simulink library "ammclib_bam"  (Simulink 9.3)
settings: Solver=VariableStepAuto  StartTime=0.0  StopTime=10.0  RelTol=1e-3
undefined symbols (not defined in the file): f16A1, f16A2, f16ADCMaxError, f16B0, f16B1, f16B2, f16C1, f16CC1, f16CC1sc, f16CC1sc_D, f16CC1sc_Q, f16CC2, f16CC2sc, f16CC2sc_D, f16CC2sc_Q, f16DerivGain, f16EGain, f16FiltCoef, f16HystOff, f16HystOn, f16IGain, f16IntegGain, f16IntegGainFW, f16IntegGainQ, f16Kd, f16Kq, f16Limit, f16LowerLimit, f16LowerLimit_D, f16LowerLimit_Q, f16LowerLimitFW, f16LowerLimitQ, f16ModIndex, f16OutValOff, f16OutValOn, f16PropGain, f16PropGainFW, f16PropGainQ, f16RampDown, f16RampUp, f16UGain, f16UpperLimit, f16UpperLimit_D, f16UpperLimit_Q, f16UpperLimitFW, f16UpperLimitQ, f16WIGain, f32A1, f32A2, f32ADCMaxError, f32B0, f32B1, f32B2, f32C1, f32CC1, f32CC1sc, f32CC1sc_D, f32CC1sc_Q, f32CC2, f32CC2sc ... (+62)
(part 8 of 15)

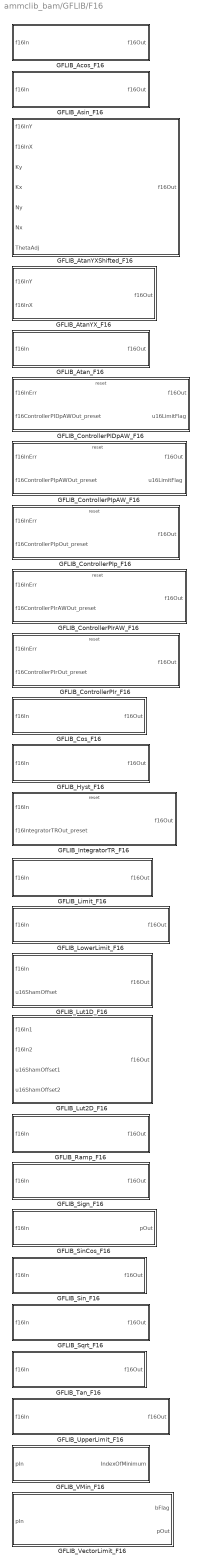
== system ammclib_bam/GFLIB/F16 ==
  GFLIB_Acos_F16 : Subsystem  TreatAsAtomicUnit=on  mask(GFLIB_Acos_F16){}
      mask help: Inverse cosine function in 16-bit fixed-point fractional implementation. Refer to the AMMCLIB User's Guide for further details.
      mask init: same as ammclib_bam/GDFLIB/F16/GDFLIB_FilterFIR_F16
      settings: RTWSystemCode=Inline
      mask Display: pos = get_param(gcb, 'Position');width = pos(3) - pos(1); height = pos(4) - pos(2);tX=width/2;tY=height - 8;color('black');text(tX,tY, 'GFLIB_Acos_F16', 'horizontalAlignment', 'center');
  GFLIB_Asin_F16 : Subsystem  TreatAsAtomicUnit=on  mask(GFLIB_Asin_F16){}
      mask help: Inverse sine function in 16-bit fixed-point fractional implementation. Refer to the AMMCLIB User's Guide for further details.
      mask init: same as ammclib_bam/GDFLIB/F16/GDFLIB_FilterFIR_F16
      settings: RTWSystemCode=Inline
      mask Display: pos = get_param(gcb, 'Position');width = pos(3) - pos(1); height = pos(4) - pos(2);tX=width/2;tY=height - 8;color('black');text(tX,tY, 'GFLIB_Asin_F16', 'horizontalAlignment', 'center');
  GFLIB_AtanYXShifted_F16 : Subsystem  TreatAsAtomicUnit=on  mask(GFLIB_AtanYXShifted_F16){}
      mask help: Shifted arctangent of two arguments Y/X in 16-bit fixed-point fractional implementation. Refer to the AMMCLIB User's Guide for further details.
      mask init: same as ammclib_bam/GDFLIB/F16/GDFLIB_FilterFIR_F16
      settings: RTWSystemCode=Inline
      mask Display: pos = get_param(gcb, 'Position');width = pos(3) - pos(1); height = pos(4) - pos(2);tX=width/2;tY=height - 8;color('black');text(tX,tY, 'GFLIB_AtanYXShifted_F16', 'horizontalAlignment', 'center');
  GFLIB_AtanYX_F16 : Subsystem  TreatAsAtomicUnit=on  mask(GFLIB_AtanYX_F16){}
      mask help: Arctangent of two arguments Y/X in 16-bit fixed-point fractional implementation. Refer to the AMMCLIB User's Guide for further details.
      mask init: same as ammclib_bam/GDFLIB/F16/GDFLIB_FilterFIR_F16
      settings: RTWSystemCode=Inline
      mask Display: pos = get_param(gcb, 'Position');width = pos(3) - pos(1); height = pos(4) - pos(2);tX=width/2;tY=height - 8;color('black');text(tX,tY, 'GFLIB_AtanYX_F16', 'horizontalAlignment', 'center');
  GFLIB_Atan_F16 : Subsystem  TreatAsAtomicUnit=on  mask(GFLIB_Atan_F16){}
      mask help: Inverse tangent function in 16-bit fixed-point fractional implementation. Refer to the AMMCLIB User's Guide for further details.
      mask init: same as ammclib_bam/GDFLIB/F16/GDFLIB_FilterFIR_F16
      settings: RTWSystemCode=Inline
      mask Display: pos = get_param(gcb, 'Position');width = pos(3) - pos(1); height = pos(4) - pos(2);tX=width/2;tY=height - 8;color('black');text(tX,tY, 'GFLIB_Atan_F16', 'horizontalAlignment', 'center');
  GFLIB_ControllerPIDpAW_F16 : Subsystem  TreatAsAtomicUnit=on  mask(GFLIB_ControllerPIDpAW_F16){showStates=Hide (faster execution), resetStatesEnable=Pre-set according to the first set of inputs after reset, f16PropGain=0, f16IntegGain=0, f16DerivGain=0, f16FiltCoef=0, s16PropGainShift=0, s16IntegGainShift=0, s16DerivGainShift=0, f16LowerLimit=0, f16UpperLimit=0}
      mask prompts: showStates "Show internal states"; resetStatesEnable "Internal state after reset"; f16PropGain "f16PropGain (Proportional gain)"; f16IntegGain "f16IntegGain (Integral gain)"; f16DerivGain "f16DerivGain (Derivative gain)"; f16FiltCoef "f16FiltCoef (Derivative term filter coefficient)"; s16PropGainShift "s16PropGainShift (Proportional gain shift)"; s16IntegGainShift "s16IntegGainShift (Integral gain shift)"; s16DerivGainShift "s16DerivGainShift (Derivative gain shift)"; f16LowerLimit "f16LowerLimit (Lower limit of the controller)"; f16UpperLimit "f16UpperLimit (Upper limit of the controller)"
      mask help: Parallel form PID controller with anti-windup in 16-bit fixed-point fractional implementation. This block supports re-initialization of the internal state during simulation. If the block is reset, the controller's output will be aligned with the input f16ControllerPIDpAWOut_preset. Refer to the AMMCLIB User's Guide for further details.
      mask init:
      | if ~evalin('base','exist(''tS8'',''var'')')
      |   if (2 ~= exist('SWLIBS_Typedefs.mat','file'))
      |       error('File SWLIBS_Typedefs.mat is not on the Matlab path. Please add the AMMCLIB "bam" folder in the Matlab Search Path.');
      |   else
      |       evalin('base', 'load(''SWLIBS_Typedefs.mat'')');
      |   end
      | end
      | if showStates == 1
      |     % hidden state variables
      |     if strcmp(get_param([gcb '/f16PropGain'], 'BlockType'), 'Inport')
      |         posblk = get_param(gcb, 'Position');
      | 
      |         pos = get_param(    [gcb, '/f16PropGain'], 'Position');
      |         orient = get_param( [gcb, '/f16PropGain'], 'Orientation');
      |         delete_block(       [gcb, '/f16PropGain']);
      |         add_block('built-in/Ground', [gcb, '/f16PropGain'], 'Position', pos, 'Orientation', orient);
      | 
      |         pos = get_param(    [gcb, '/f16IntegGain'], 'Position');
      |         orient = get_param( [gcb, '/f16IntegGain'], 'Orientation');
      |         delete_block(       [gcb, '/f16IntegGain']);
      |         add_block('built-in/Ground', [gcb, '/f16IntegGain'], 'Position', pos, 'Orientation', orient);
      | 
      |         pos = get_param(    [gcb, '/f16DerivGain'], 'Position');
      |         orient = get_param( [gcb, '/f16DerivGain'], 'Orientation');
      |         delete_block(       [gcb, '/f16DerivGain']);
      |         add_block('built-in/Ground', [gcb, '/f16DerivGain'], 'Position', pos, 'Orientation', orient);
      | 
      |         pos = get_param(    [gcb, '/f16FiltCoef'], 'Position');
      |         orient = get_param( [gcb, '/f16FiltCoef'], 'Orientation');
      |         delete_block(       [gcb, '/f16FiltCoef']);
      |         add_block('built-in/Ground', [gcb, '/f16FiltCoef'], 'Position', pos, 'Orientation', orient);
      | 
      |         pos = get_param(    [gcb, '/s16PropGainShift'], 'Position');
      |         orient = get_param( [gcb, '/s16PropGainShift'], 'Orientation');
      |         delete_block(       [gcb, '/s16PropGainShift']);
      |         add_block('built-in/Ground', [gcb, '/s16PropGainShift'], 'Position', pos, 'Orientation', orient);
      | 
      |         pos = get_param(    [gcb, '/s16IntegGainShift'], 'Position');
      |         orient = get_param( [gcb, '/s16IntegGainShift'], 'Orientation');
      |         delete_block(       [gcb, '/s16IntegGainShift']);
      |         add_block('built-in/Ground', [gcb, '/s16IntegGainShift'], 'Position', pos, 'Orientation', orient);
      | 
      |         pos = get_param(    [gcb, '/s16DerivGainShift'], 'Position');
      |         orient = get_param( [gcb, '/s16DerivGainShift'], 'Orientation');
      |         delete_block(       [gcb, '/s16DerivGainShift']);
      |         add_block('built-in/Ground', [gcb, '/s16DerivGainShift'], 'Position', pos, 'Orientation', orient);
      | 
      |         pos = get_param(    [gcb, '/f16LowerLimit'], 'Position');
      |         orient = get_param( [gcb, '/f16LowerLimit'], 'Orientation');
      |         delete_block(       [gcb, '/f16LowerLimit']);
      |         add_block('built-in/Ground', [gcb, '/f16LowerLimit'], 'Position', pos, 'Orientation', orient);
      | 
      |         pos = get_param(    [gcb, '/f16UpperLimit'], 'Position');
      |         orient = get_param( [gcb, '/f16UpperLimit'], 'Orientation');
      |         delete_block(       [gcb, '/f16UpperLimit']);
      |         add_block('built-in/Ground', [gcb, '/f16UpperLimit'], 'Position', pos, 'Orientation', orient);
      | 
      |         pos = get_param(    [gcb, '/f32IntegPartK_1'], 'Position');
      |         orient = get_param( [gcb, '/f32IntegPartK_1'], 'Orientation');
      |         delete_block(       [gcb, '/f32IntegPartK_1']);
      |         add_block('built-in/Ground', [gcb, '/f32IntegPartK_1'], 'Position', pos, 'Orientation', orient);
      | 
      |         pos = get_param(    [gcb, '/f16DerivPartK_1'], 'Position');
      |         orient = get_param( [gcb, '/f16DerivPartK_1'], 'Orientation');
      |         delete_block(       [gcb, '/f16DerivPartK_1']);
      |         add_block('built-in/Ground', [gcb, '/f16DerivPartK_1'], 'Position', pos, 'Orientation', orient);
      | 
      |         pos = get_param(    [gcb, '/f16InK_1'], 'Position');
      |         orient = get_param( [gcb, '/f16InK_1'], 'Orientation');
      |         delete_block(       [gcb, '/f16InK_1']);
      |         add_block('built-in/Ground', [gcb, '/f16InK_1'], 'Position', pos, 'Orientation', orient);
      | 
      | 
      |         pos = get_param(    [gcb '/f32IntegPartK_1_Out'], 'Position');
      |         orient = get_param( [gcb '/f32IntegPartK_1_Out'], 'Orientation');
      |         delete_block(       [gcb '/f32IntegPartK_1_Out']);
      |         add_block('built-in/Terminator', [gcb '/f32IntegPartK_1_Out'], 'Position', pos, 'Orientation', orient);
      | 
      |         pos = get_param(    [gcb '/f16DerivPartK_1_Out'], 'Position');
      |         orient = get_param( [gcb '/f16DerivPartK_1_Out'], 'Orientation');
      |         delete_block(       [gcb '/f16DerivPartK_1_Out']);
      |         add_block('built-in/Terminator', [gcb '/f16DerivPartK_1_Out'], 'Position', pos, 'Orientation', orient);
      | 
      |         pos = get_param(    [gcb '/f16InK_1_Out'], 'Position');
      |         orient = get_param( [gcb '/f16InK_1_Out'], 'Orientation');
      |         delete_block(       [gcb '/f16InK_1_Out']);
      |         add_block('built-in/Terminator', [gcb '/f16InK_1_Out'], 'Position', pos, 'Orientation', orient);
      | 
      | 
      |         set_param([gcb '/f16InErr'], 'Port', '1');
      |         set_param([gcb '/f16ControllerPIDpAWOut_preset'], 'Port', '2');
      | 
      |         set_param([gcb '/f16Out'], 'Port', '1');
      |         set_param([gcb '/u16LimitFlag'], 'Port', '2');
      | 
      |         set_param(gcb,'MaskEnables',{'on','on','on','on','on','on','on','on','on','on','on'});
      | 
      |         if (posblk(4) - posblk(2)) > 75
      |           height = 75;
      |           set_param(gcb,'Position',[posblk(1), posblk(2), posblk(3), posblk(2)+height])
      |         end
      |     end
      | else
      |     % shown state variables
      |     if strcmp(get_param([gcb '/f16PropGain'], 'BlockType'), 'Ground')
      |         posblk = get_param(gcb, 'Position');
      | 
      |         pos = get_param(    [gcb, '/f16PropGain'], 'Position');
      |         orient = get_param( [gcb, '/f16PropGain'], 'Orientation');
      |         delete_block(       [gcb, '/f16PropGain']);
      |         add_block('built-in/Inport', [gcb, '/f16PropGain'], 'Position', pos, 'Orientation', orient, 'OutDataTypeStr', 'int16');
      | 
      |         pos = get_param(    [gcb, '/f16IntegGain'], 'Position');
      |         orient = get_param( [gcb, '/f16IntegGain'], 'Orientation');
      |         delete_block(       [gcb, '/f16IntegGain']);
      |         add_block('built-in/Inport', [gcb, '/f16IntegGain'], 'Position', pos, 'Orientation', orient, 'OutDataTypeStr', 'int16');
      | 
      |         pos = get_param(    [gcb, '/f16DerivGain'], 'Position');
      |         orient = get_param( [gcb, '/f16DerivGain'], 'Orientation');
      |         delete_block(       [gcb, '/f16DerivGain']);
      |         add_block('built-in/Inport', [gcb, '/f16DerivGain'], 'Position', pos, 'Orientation', orient, 'OutDataTypeStr', 'int16');
      | 
      |         pos = get_param(    [gcb, '/f16FiltCoef'], 'Position');
      |         orient = get_param( [gcb, '/f16FiltCoef'], 'Orientation');
      |         delete_block(       [gcb, '/f16FiltCoef']);
      |         add_block('built-in/Inport', [gcb, '/f16FiltCoef'], 'Position', pos, 'Orientation', orient, 'OutDataTypeStr', 'int16');
      | 
      |         pos = get_param(    [gcb, '/s16PropGainShift'], 'Position');
      |         orient = get_param( [gcb, '/s16PropGainShift'], 'Orientation');
      |         delete_block(       [gcb, '/s16PropGainShift']);
      |         add_block('built-in/Inport', [gcb, '/s16PropGainShift'], 'Position', pos, 'Orientation', orient, 'OutDataTypeStr', 'int16');
      | 
      |         pos = get_param(    [gcb, '/s16IntegGainShift'], 'Position');
      |         orient = get_param( [gcb, '/s16IntegGainShift'], 'Orientation');
      |         delete_block(       [gcb, '/s16IntegGainShift']);
      |         add_block('built-in/Inport', [gcb, '/s16IntegGainShift'], 'Position', pos, 'Orientation', orient, 'OutDataTypeStr', 'int16');
      | 
      |         pos = get_param(    [gcb, '/s16DerivGainShift'], 'Position');
      |         orient = get_param( [gcb, '/s16DerivGainShift'], 'Orientation');
      |         delete_block(       [gcb, '/s16DerivGainShift']);
      |         add_block('built-in/Inport', [gcb, '/s16DerivGainShift'], 'Position', pos, 'Orientation', orient, 'OutDataTypeStr', 'int16');
      | 
      |         pos = get_param(    [gcb, '/f16LowerLimit'], 'Position');
      |         orient = get_param( [gcb, '/f16LowerLimit'], 'Orientation');
      |         delete_block(       [gcb, '/f16LowerLimit']);
      |         add_block('built-in/Inport', [gcb, '/f16LowerLimit'], 'Position', pos, 'Orientation', orient, 'OutDataTypeStr', 'int16');
      | 
      |         pos = get_param(    [gcb, '/f16UpperLimit'], 'Position');
      |         orient = get_param( [gcb, '/f16UpperLimit'], 'Orientation');
      |         delete_block(       [gcb, '/f16UpperLimit']);
      |         add_block('built-in/Inport', [gcb, '/f16UpperLimit'], 'Position', pos, 'Orientation', orient, 'OutDataTypeStr', 'int16');
      | 
      |         pos = get_param(    [gcb, '/f32IntegPartK_1'], 'Position');
      |         orient = get_param( [gcb, '/f32IntegPartK_1'], 'Orientation');
      |         delete_block(       [gcb, '/f32IntegPartK_1']);
      |         add_block('built-in/Inport', [gcb, '/f32IntegPartK_1'], 'Position', pos, 'Orientation', orient, 'OutDataTypeStr', 'int32');
      | 
      |         pos = get_param(    [gcb, '/f16DerivPartK_1'], 'Position');
      |         orient = get_param( [gcb, '/f16DerivPartK_1'], 'Orientation');
      |         delete_block(       [gcb, '/f16DerivPartK_1']);
      |         add_block('built-in/Inport', [gcb, '/f16DerivPartK_1'], 'Position', pos, 'Orientation', orient, 'OutDataTypeStr', 'int16');
      | 
      |         pos = get_param(    [gcb, '/f16InK_1'], 'Position');
      |         orient = get_param( [gcb, '/f16InK_1'], 'Orientation');
      |         delete_block(       [gcb, '/f16InK_1']);
      |         add_block('built-in/Inport', [gcb, '/f16InK_1'], 'Position', pos, 'Orientation', orient, 'OutDataTypeStr', 'int16');
      | 
      | 
      |         pos = get_param(    [gcb '/f32IntegPartK_1_Out'], 'Position');
      |         orient = get_param( [gcb '/f32IntegPartK_1_Out'], 'Orientation');
      |         delete_block(       [gcb '/f32IntegPartK_1_Out']);
      |         add_block('built-in/Outport', [gcb '/f32IntegPartK_1_Out'], 'Position', pos, 'Orientation', orient);
      | 
      |         pos = get_param(    [gcb '/f16DerivPartK_1_Out'], 'Position');
      |         orient = get_param( [gcb '/f16DerivPartK_1_Out'], 'Orientation');
      |         delete_block(       [gcb '/f16DerivPartK_1_Out']);
      |         add_block('built-in/Outport', [gcb '/f16DerivPartK_1_Out'], 'Position', pos, 'Orientation', orient);
      | 
      |         pos = get_param(    [gcb '/f16InK_1_Out'], 'Position');
      |         orient = get_param( [gcb '/f16InK_1_Out'], 'Orientation');
      |         delete_block(       [gcb '/f16InK_1_Out']);
      |         add_block('built-in/Outport', [gcb '/f16InK_1_Out'], 'Position', pos, 'Orientation', orient);
      | 
      | 
      |         set_param([gcb '/f16InErr'], 'Port', '1');
      |         set_param([gcb '/f16ControllerPIDpAWOut_preset'], 'Port', '2');
      |         set_param([gcb '/f16PropGain'], 'Port', '3');
      |         set_param([gcb '/f16IntegGain'], 'Port', '4');
      |         set_param([gcb '/f16DerivGain'], 'Port', '5');
      |         set_param([gcb '/f16FiltCoef'], 'Port', '6');
      |         set_param([gcb '/s16PropGainShift'], 'Port', '7');
      |         set_param([gcb '/s16IntegGainShift'], 'Port', '8');
      |         set_param([gcb '/s16DerivGainShift'], 'Port', '9');
      |         set_param([gcb '/f16LowerLimit'], 'Port', '10');
      |         set_param([gcb '/f16UpperLimit'], 'Port', '11');
      |         set_param([gcb '/f32IntegPartK_1'], 'Port', '12');
      |         set_param([gcb '/f16DerivPartK_1'], 'Port', '13');
      |         set_param([gcb '/f16InK_1'], 'Port', '14');
      | 
      |         set_param([gcb '/f16Out'], 'Port', '1');
      |         set_param([gcb '/u16LimitFlag'], 'Port', '2');
      |         set_param([gcb '/f32IntegPartK_1_Out'], 'Port', '3');
      |         set_param([gcb '/f16DerivPartK_1_Out'], 'Port', '4');
      |         set_param([gcb '/f16InK_1_Out'], 'Port', '5');
      | 
      |         set_param(gcb,'MaskEnables',{'on','on','off','off','off','off','off','off','off','off','off'});
      | 
      |         if (posblk(4) - posblk(2)) < 375
      |           height = 375;
      |           set_param(gcb,'Position',[posblk(1), posblk(2), posblk(3), posblk(2)+height])
      |         end
      |     end
      | end
      settings: RTWSystemCode=Inline
      mask TypeOptions showStates: Hide (faster execution) | Show (allows debugging; connect feedback loops manually)
      mask Callback showStates:
      | maskStr = get_param(gcb,'showStates');
      | if strcmp(maskStr,'Hide (faster execution)'),
      |     set_param(gcb,'MaskEnables',{'on','on','on','on','on','on','on','on','on','on','on'});
      | else
      |     set_param(gcb,'MaskEnables',{'on','on','off','off','off','off','off','off','off','off','off'});
      | end
      mask TypeOptions resetStatesEnable: Pre-set according to the first set of inputs after reset | Clear to zero
      mask Display:
      | color('black');
      | pos = get_param(gcb, 'Position');
      | width = pos(3) - pos(1);
      | height = pos(4) - pos(2);
      | tX=width/2;
      | tY=height - 25;
      | color('black');
      | text(tX,tY, 'GFLIB_ControllerPIDpAW_F16', 'horizontalAlignment', 'center');
      | if showStates == 2
      |   color('red');
      |   text(tX,tY - 20, ['debugging mode' char(13) char(10) '(limited performance)'], 'horizontalAlignment', 'center');
      | end
  GFLIB_ControllerPIpAW_F16 : Subsystem  TreatAsAtomicUnit=on  mask(GFLIB_ControllerPIpAW_F16){showStates=Hide (faster execution), resetStatesEnable=Pre-set according to the first set of inputs after reset, f16PropGain=0, f16IntegGain=0, s16PropGainShift=0, s16IntegGainShift=0, f16LowerLimit=0, f16UpperLimit=0}
      mask prompts: showStates "Show internal states"; resetStatesEnable "Internal state after reset"; f16PropGain "f16PropGain (Proportional gain)"; f16IntegGain "f16IntegGain (Integral gain)"; s16PropGainShift "s16PropGainShift (Proportional gain shift)"; s16IntegGainShift "s16IntegGainShift (Integral gain shift)"; f16LowerLimit "f16LowerLimit (Lower limit of the controller)"; f16UpperLimit "f16UpperLimit (Upper limit of the controller)"
      mask help: Parallel form PI controller with anti-windup in 16-bit fixed-point fractional implementation. This block supports re-initialization of the internal state during simulation. If the block is reset, the controller's output will be aligned with the input f16ControllerPIpAWOut_preset. Refer to the AMMCLIB User's Guide for further details.
      mask init:
      | if ~evalin('base','exist(''tS8'',''var'')')
      |   if (2 ~= exist('SWLIBS_Typedefs.mat','file'))
      |       error('File SWLIBS_Typedefs.mat is not on the Matlab path. Please add the AMMCLIB "bam" folder in the Matlab Search Path.');
      |   else
      |       evalin('base', 'load(''SWLIBS_Typedefs.mat'')');
      |   end
      | end
      | if showStates == 1
      |     % hidden state variables
      |     if strcmp(get_param([gcb '/f16PropGain'], 'BlockType'), 'Inport')
      |         posblk = get_param(gcb, 'Position');
      | 
      |         pos = get_param(    [gcb, '/f16PropGain'], 'Position');
      |         orient = get_param( [gcb, '/f16PropGain'], 'Orientation');
      |         delete_block(       [gcb, '/f16PropGain']);
      |         add_block('built-in/Ground', [gcb, '/f16PropGain'], 'Position', pos, 'Orientation', orient);
      | 
      |         pos = get_param(    [gcb, '/f16IntegGain'], 'Position');
      |         orient = get_param( [gcb, '/f16IntegGain'], 'Orientation');
      |         delete_block(       [gcb, '/f16IntegGain']);
      |         add_block('built-in/Ground', [gcb, '/f16IntegGain'], 'Position', pos, 'Orientation', orient);
      | 
      |         pos = get_param(    [gcb, '/s16PropGainShift'], 'Position');
      |         orient = get_param( [gcb, '/s16PropGainShift'], 'Orientation');
      |         delete_block(       [gcb, '/s16PropGainShift']);
      |         add_block('built-in/Ground', [gcb, '/s16PropGainShift'], 'Position', pos, 'Orientation', orient);
      | 
      |         pos = get_param(    [gcb, '/s16IntegGainShift'], 'Position');
      |         orient = get_param( [gcb, '/s16IntegGainShift'], 'Orientation');
      |         delete_block(       [gcb, '/s16IntegGainShift']);
      |         add_block('built-in/Ground', [gcb, '/s16IntegGainShift'], 'Position', pos, 'Orientation', orient);
      | 
      |         pos = get_param(    [gcb, '/f16LowerLimit'], 'Position');
      |         orient = get_param( [gcb, '/f16LowerLimit'], 'Orientation');
      |         delete_block(       [gcb, '/f16LowerLimit']);
      |         add_block('built-in/Ground', [gcb, '/f16LowerLimit'], 'Position', pos, 'Orientation', orient);
      | 
      |         pos = get_param(    [gcb, '/f16UpperLimit'], 'Position');
      |         orient = get_param( [gcb, '/f16UpperLimit'], 'Orientation');
      |         delete_block(       [gcb, '/f16UpperLimit']);
      |         add_block('built-in/Ground', [gcb, '/f16UpperLimit'], 'Position', pos, 'Orientation', orient);
      | 
      |         pos = get_param(    [gcb, '/f32IntegPartK_1'], 'Position');
      |         orient = get_param( [gcb, '/f32IntegPartK_1'], 'Orientation');
      |         delete_block(       [gcb, '/f32IntegPartK_1']);
      |         add_block('built-in/Ground', [gcb, '/f32IntegPartK_1'], 'Position', pos, 'Orientation', orient);
      | 
      |         pos = get_param(    [gcb, '/f16InK_1'], 'Position');
      |         orient = get_param( [gcb, '/f16InK_1'], 'Orientation');
      |         delete_block(       [gcb, '/f16InK_1']);
      |         add_block('built-in/Ground', [gcb, '/f16InK_1'], 'Position', pos, 'Orientation', orient);
      | 
      | 
      |         pos = get_param(    [gcb '/f32IntegPartK_1_Out'], 'Position');
      |         orient = get_param( [gcb '/f32IntegPartK_1_Out'], 'Orientation');
      |         delete_block(       [gcb '/f32IntegPartK_1_Out']);
      |         add_block('built-in/Terminator', [gcb '/f32IntegPartK_1_Out'], 'Position', pos, 'Orientation', orient);
      | 
      |         pos = get_param(    [gcb '/f16InK_1_Out'], 'Position');
      |         orient = get_param( [gcb '/f16InK_1_Out'], 'Orientation');
      |         delete_block(       [gcb '/f16InK_1_Out']);
      |         add_block('built-in/Terminator', [gcb '/f16InK_1_Out'], 'Position', pos, 'Orientation', orient);
      | 
      | 
      |         set_param([gcb '/f16InErr'], 'Port', '1');
      |         set_param([gcb '/f16ControllerPIpAWOut_preset'], 'Port', '2');
      | 
      |         set_param([gcb '/f16Out'], 'Port', '1');
      |         set_param([gcb '/u16LimitFlag'], 'Port', '2');
      | 
      |         set_param(gcb,'MaskEnables',{'on','on','on','on','on','on','on','on'});
      | 
      |         if (posblk(4) - posblk(2)) > 75
      |           height = 75;
      |           set_param(gcb,'Position',[posblk(1), posblk(2), posblk(3), posblk(2)+height])
      |         end
      |     end
      | else
      |     % shown state variables
      |     if strcmp(get_param([gcb '/f16PropGain'], 'BlockType'), 'Ground')
      |         posblk = get_param(gcb, 'Position');
      | 
      |         pos = get_param(    [gcb, '/f16PropGain'], 'Position');
      |         orient = get_param( [gcb, '/f16PropGain'], 'Orientation');
      |         delete_block(       [gcb, '/f16PropGain']);
      |         add_block('built-in/Inport', [gcb, '/f16PropGain'], 'Position', pos, 'Orientation', orient, 'OutDataTypeStr', 'int16');
      | 
      |         pos = get_param(    [gcb, '/f16IntegGain'], 'Position');
      |         orient = get_param( [gcb, '/f16IntegGain'], 'Orientation');
      |         delete_block(       [gcb, '/f16IntegGain']);
      |         add_block('built-in/Inport', [gcb, '/f16IntegGain'], 'Position', pos, 'Orientation', orient, 'OutDataTypeStr', 'int16');
      | 
      |         pos = get_param(    [gcb, '/s16PropGainShift'], 'Position');
      |         orient = get_param( [gcb, '/s16PropGainShift'], 'Orientation');
      |         delete_block(       [gcb, '/s16PropGainShift']);
      |         add_block('built-in/Inport', [gcb, '/s16PropGainShift'], 'Position', pos, 'Orientation', orient, 'OutDataTypeStr', 'int16');
      | 
      |         pos = get_param(    [gcb, '/s16IntegGainShift'], 'Position');
      |         orient = get_param( [gcb, '/s16IntegGainShift'], 'Orientation');
      |         delete_block(       [gcb, '/s16IntegGainShift']);
      |         add_block('built-in/Inport', [gcb, '/s16IntegGainShift'], 'Position', pos, 'Orientation', orient, 'OutDataTypeStr', 'int16');
      | 
      |         pos = get_param(    [gcb, '/f16LowerLimit'], 'Position');
      |         orient = get_param( [gcb, '/f16LowerLimit'], 'Orientation');
      |         delete_block(       [gcb, '/f16LowerLimit']);
      |         add_block('built-in/Inport', [gcb, '/f16LowerLimit'], 'Position', pos, 'Orientation', orient, 'OutDataTypeStr', 'int16');
      | 
      |         pos = get_param(    [gcb, '/f16UpperLimit'], 'Position');
      |         orient = get_param( [gcb, '/f16UpperLimit'], 'Orientation');
      |         delete_block(       [gcb, '/f16UpperLimit']);
      |         add_block('built-in/Inport', [gcb, '/f16UpperLimit'], 'Position', pos, 'Orientation', orient, 'OutDataTypeStr', 'int16');
      | 
      |         pos = get_param(    [gcb, '/f32IntegPartK_1'], 'Position');
      |         orient = get_param( [gcb, '/f32IntegPartK_1'], 'Orientation');
      |         delete_block(       [gcb, '/f32IntegPartK_1']);
      |         add_block('built-in/Inport', [gcb, '/f32IntegPartK_1'], 'Position', pos, 'Orientation', orient, 'OutDataTypeStr', 'int32');
      | 
      |         pos = get_param(    [gcb, '/f16InK_1'], 'Position');
      |         orient = get_param( [gcb, '/f16InK_1'], 'Orientation');
      |         delete_block(       [gcb, '/f16InK_1']);
      |         add_block('built-in/Inport', [gcb, '/f16InK_1'], 'Position', pos, 'Orientation', orient, 'OutDataTypeStr', 'int16');
      | 
      | 
      |         pos = get_param(    [gcb '/f32IntegPartK_1_Out'], 'Position');
      |         orient = get_param( [gcb '/f32IntegPartK_1_Out'], 'Orientation');
      |         delete_block(       [gcb '/f32IntegPartK_1_Out']);
      |         add_block('built-in/Outport', [gcb '/f32IntegPartK_1_Out'], 'Position', pos, 'Orientation', orient);
      | 
      |         pos = get_param(    [gcb '/f16InK_1_Out'], 'Position');
      |         orient = get_param( [gcb '/f16InK_1_Out'], 'Orientation');
      |         delete_block(       [gcb '/f16InK_1_Out']);
      |         add_block('built-in/Outport', [gcb '/f16InK_1_Out'], 'Position', pos, 'Orientation', orient);
      | 
      | 
      |         set_param([gcb '/f16InErr'], 'Port', '1');
      |         set_param([gcb '/f16ControllerPIpAWOut_preset'], 'Port', '2');
      |         set_param([gcb '/f16PropGain'], 'Port', '3');
      |         set_param([gcb '/f16IntegGain'], 'Port', '4');
      |         set_param([gcb '/s16PropGainShift'], 'Port', '5');
      |         set_param([gcb '/s16IntegGainShift'], 'Port', '6');
      |         set_param([gcb '/f16LowerLimit'], 'Port', '7');
      |         set_param([gcb '/f16UpperLimit'], 'Port', '8');
      |         set_param([gcb '/f32IntegPartK_1'], 'Port', '9');
      |         set_param([gcb '/f16InK_1'], 'Port', '10');
      | 
      |         set_param([gcb '/f16Out'], 'Port', '1');
      |         set_param([gcb '/u16LimitFlag'], 'Port', '2');
      |         set_param([gcb '/f32IntegPartK_1_Out'], 'Port', '3');
      |         set_param([gcb '/f16InK_1_Out'], 'Port', '4');
      | 
      |         set_param(gcb,'MaskEnables',{'on','on','off','off','off','off','off','off'});
      | 
      |         if (posblk(4) - posblk(2)) < 275
      |           height = 275;
      |           set_param(gcb,'Position',[posblk(1), posblk(2), posblk(3), posblk(2)+height])
      |         end
      |     end
      | end
      settings: RTWSystemCode=Inline
      mask TypeOptions showStates: Hide (faster execution) | Show (allows debugging; connect feedback loops manually)
      mask Callback showStates:
      | maskStr = get_param(gcb,'showStates');
      | if strcmp(maskStr,'Hide (faster execution)'),
      |     set_param(gcb,'MaskEnables',{'on','on','on','on','on','on','on','on'});
      | else
      |     set_param(gcb,'MaskEnables',{'on','on','off','off','off','off','off','off'});
      | end
      mask TypeOptions resetStatesEnable: Pre-set according to the first set of inputs after reset | Clear to zero
      mask Display:
      | color('black');
      | pos = get_param(gcb, 'Position');
      | width = pos(3) - pos(1);
      | height = pos(4) - pos(2);
      | tX=width/2;
      | tY=height - 25;
      | color('black');
      | text(tX,tY, 'GFLIB_ControllerPIpAW_F16', 'horizontalAlignment', 'center');
      | if showStates == 2
      |   color('red');
      |   text(tX,tY - 20, ['debugging mode' char(13) char(10) '(limited performance)'], 'horizontalAlignment', 'center');
      | end
  GFLIB_ControllerPIp_F16 : Subsystem  TreatAsAtomicUnit=on  mask(GFLIB_ControllerPIp_F16){showStates=Hide (faster execution), resetStatesEnable=Pre-set according to the first set of inputs after reset, f16PropGain=0, f16IntegGain=0, s16PropGainShift=0, s16IntegGainShift=0}
      mask prompts: showStates "Show internal states"; resetStatesEnable "Internal state after reset"; f16PropGain "f16PropGain (Proportional gain)"; f16IntegGain "f16IntegGain (Integral gain)"; s16PropGainShift "s16PropGainShift (Proportional gain shift)"; s16IntegGainShift "s16IntegGainShift (Integral gain shift)"
      mask help: Parallel form PI controller without anti-windup in 16-bit fixed-point fractional implementation. This block supports re-initialization of the internal state during simulation. If the block is reset, the controller's output will be aligned with the input f16ControllerPIpOut_preset. Refer to the AMMCLIB User's Guide for further details.
      mask init:
      | if ~evalin('base','exist(''tS8'',''var'')')
      |   if (2 ~= exist('SWLIBS_Typedefs.mat','file'))
      |       error('File SWLIBS_Typedefs.mat is not on the Matlab path. Please add the AMMCLIB "bam" folder in the Matlab Search Path.');
      |   else
      |       evalin('base', 'load(''SWLIBS_Typedefs.mat'')');
      |   end
      | end
      | if showStates == 1
      |     % hidden state variables
      |     if strcmp(get_param([gcb '/f16PropGain'], 'BlockType'), 'Inport')
      |         posblk = get_param(gcb, 'Position');
      | 
      |         pos = get_param(    [gcb, '/f16PropGain'], 'Position');
      |         orient = get_param( [gcb, '/f16PropGain'], 'Orientation');
      |         delete_block(       [gcb, '/f16PropGain']);
      |         add_block('built-in/Ground', [gcb, '/f16PropGain'], 'Position', pos, 'Orientation', orient);
      | 
      |         pos = get_param(    [gcb, '/f16IntegGain'], 'Position');
      |         orient = get_param( [gcb, '/f16IntegGain'], 'Orientation');
      |         delete_block(       [gcb, '/f16IntegGain']);
      |         add_block('built-in/Ground', [gcb, '/f16IntegGain'], 'Position', pos, 'Orientation', orient);
      | 
      |         pos = get_param(    [gcb, '/s16PropGainShift'], 'Position');
      |         orient = get_param( [gcb, '/s16PropGainShift'], 'Orientation');
      |         delete_block(       [gcb, '/s16PropGainShift']);
      |         add_block('built-in/Ground', [gcb, '/s16PropGainShift'], 'Position', pos, 'Orientation', orient);
      | 
      |         pos = get_param(    [gcb, '/s16IntegGainShift'], 'Position');
      |         orient = get_param( [gcb, '/s16IntegGainShift'], 'Orientation');
      |         delete_block(       [gcb, '/s16IntegGainShift']);
      |         add_block('built-in/Ground', [gcb, '/s16IntegGainShift'], 'Position', pos, 'Orientation', orient);
      | 
      |         pos = get_param(    [gcb, '/f32IntegPartK_1'], 'Position');
      |         orient = get_param( [gcb, '/f32IntegPartK_1'], 'Orientation');
      |         delete_block(       [gcb, '/f32IntegPartK_1']);
      |         add_block('built-in/Ground', [gcb, '/f32IntegPartK_1'], 'Position', pos, 'Orientation', orient);
      | 
      |         pos = get_param(    [gcb, '/f16InK_1'], 'Position');
      |         orient = get_param( [gcb, '/f16InK_1'], 'Orientation');
      |         delete_block(       [gcb, '/f16InK_1']);
      |         add_block('built-in/Ground', [gcb, '/f16InK_1'], 'Position', pos, 'Orientation', orient);
      | 
      | 
      |         pos = get_param(    [gcb '/f32IntegPartK_1_Out'], 'Position');
      |         orient = get_param( [gcb '/f32IntegPartK_1_Out'], 'Orientation');
      |         delete_block(       [gcb '/f32IntegPartK_1_Out']);
      |         add_block('built-in/Terminator', [gcb '/f32IntegPartK_1_Out'], 'Position', pos, 'Orientation', orient);
      | 
      |         pos = get_param(    [gcb '/f16InK_1_Out'], 'Position');
      |         orient = get_param( [gcb '/f16InK_1_Out'], 'Orientation');
      |         delete_block(       [gcb '/f16InK_1_Out']);
      |         add_block('built-in/Terminator', [gcb '/f16InK_1_Out'], 'Position', pos, 'Orientation', orient);
      | 
      | 
      |         set_param([gcb '/f16InErr'], 'Port', '1');
      |         set_param([gcb '/f16ControllerPIpOut_preset'], 'Port', '2');
      | 
      |         set_param([gcb '/f16Out'], 'Port', '1');
      | 
      |         set_param(gcb,'MaskEnables',{'on','on','on','on','on','on'});
      | 
      |         if (posblk(4) - posblk(2)) > 75
      |           height = 75;
      |           set_param(gcb,'Position',[posblk(1), posblk(2), posblk(3), posblk(2)+height])
      |         end
      |     end
      | else
      |     % shown state variables
      |     if strcmp(get_param([gcb '/f16PropGain'], 'BlockType'), 'Ground')
      |         posblk = get_param(gcb, 'Position');
      | 
      |         pos = get_param(    [gcb, '/f16PropGain'], 'Position');
      |         orient = get_param( [gcb, '/f16PropGain'], 'Orientation');
      |         delete_block(       [gcb, '/f16PropGain']);
      |         add_block('built-in/Inport', [gcb, '/f16PropGain'], 'Position', pos, 'Orientation', orient, 'OutDataTypeStr', 'int16');
      | 
      |         pos = get_param(    [gcb, '/f16IntegGain'], 'Position');
      |         orient = get_param( [gcb, '/f16IntegGain'], 'Orientation');
      |         delete_block(       [gcb, '/f16IntegGain']);
      |         add_block('built-in/Inport', [gcb, '/f16IntegGain'], 'Position', pos, 'Orientation', orient, 'OutDataTypeStr', 'int16');
      | 
      |         pos = get_param(    [gcb, '/s16PropGainShift'], 'Position');
      |         orient = get_param( [gcb, '/s16PropGainShift'], 'Orientation');
      |         delete_block(       [gcb, '/s16PropGainShift']);
      |         add_block('built-in/Inport', [gcb, '/s16PropGainShift'], 'Position', pos, 'Orientation', orient, 'OutDataTypeStr', 'int16');
      | 
      |         pos = get_param(    [gcb, '/s16IntegGainShift'], 'Position');
      |         orient = get_param( [gcb, '/s16IntegGainShift'], 'Orientation');
      |         delete_block(       [gcb, '/s16IntegGainShift']);
      |         add_block('built-in/Inport', [gcb, '/s16IntegGainShift'], 'Position', pos, 'Orientation', orient, 'OutDataTypeStr', 'int16');
      | 
      |         pos = get_param(    [gcb, '/f32IntegPartK_1'], 'Position');
      |         orient = get_param( [gcb, '/f32IntegPartK_1'], 'Orientation');
      |         delete_block(       [gcb, '/f32IntegPartK_1']);
      |         add_block('built-in/Inport', [gcb, '/f32IntegPartK_1'], 'Position', pos, 'Orientation', orient, 'OutDataTypeStr', 'int32');
      | 
      |         pos = get_param(    [gcb, '/f16InK_1'], 'Position');
      |         orient = get_param( [gcb, '/f16InK_1'], 'Orientation');
      |         delete_block(       [gcb, '/f16InK_1']);
      |         add_block('built-in/Inport', [gcb, '/f16InK_1'], 'Position', pos, 'Orientation', orient, 'OutDataTypeStr', 'int16');
      | 
      | 
      |         pos = get_param(    [gcb '/f32IntegPartK_1_Out'], 'Position');
      |         orient = get_param( [gcb '/f32IntegPartK_1_Out'], 'Orientation');
      |         delete_block(       [gcb '/f32IntegPartK_1_Out']);
      |         add_block('built-in/Outport', [gcb '/f32IntegPartK_1_Out'], 'Position', pos, 'Orientation', orient);
      | 
      |         pos = get_param(    [gcb '/f16InK_1_Out'], 'Position');
      |         orient = get_param( [gcb '/f16InK_1_Out'], 'Orientation');
      |         delete_block(       [gcb '/f16InK_1_Out']);
      |         add_block('built-in/Outport', [gcb '/f16InK_1_Out'], 'Position', pos, 'Orientation', orient);
      | 
      | 
      |         set_param([gcb '/f16InErr'], 'Port', '1');
      |         set_param([gcb '/f16ControllerPIpOut_preset'], 'Port', '2');
      |         set_param([gcb '/f16PropGain'], 'Port', '3');
      |         set_param([gcb '/f16IntegGain'], 'Port', '4');
      |         set_param([gcb '/s16PropGainShift'], 'Port', '5');
      |         set_param([gcb '/s16IntegGainShift'], 'Port', '6');
      |         set_param([gcb '/f32IntegPartK_1'], 'Port', '7');
      |         set_param([gcb '/f16InK_1'], 'Port', '8');
      | 
      |         set_param([gcb '/f16Out'], 'Port', '1');
      |         set_param([gcb '/f32IntegPartK_1_Out'], 'Port', '2');
      |         set_param([gcb '/f16InK_1_Out'], 'Port', '3');
      | 
      |         set_param(gcb,'MaskEnables',{'on','on','off','off','off','off'});
      | 
      |         if (posblk(4) - posblk(2)) < 225
      |           height = 225;
      |           set_param(gcb,'Position',[posblk(1), posblk(2), posblk(3), posblk(2)+height])
      |         end
      |     end
      | end
      settings: RTWSystemCode=Inline
      mask TypeOptions showStates: Hide (faster execution) | Show (allows debugging; connect feedback loops manually)
      mask Callback showStates:
      | maskStr = get_param(gcb,'showStates');
      | if strcmp(maskStr,'Hide (faster execution)'),
      |     set_param(gcb,'MaskEnables',{'on','on','on','on','on','on'});
      | else
      |     set_param(gcb,'MaskEnables',{'on','on','off','off','off','off'});
      | end
      mask TypeOptions resetStatesEnable: Pre-set according to the first set of inputs after reset | Clear to zero
      mask Display:
      | color('black');
      | pos = get_param(gcb, 'Position');
      | width = pos(3) - pos(1);
      | height = pos(4) - pos(2);
      | tX=width/2;
      | tY=height - 25;
      | color('black');
      | text(tX,tY, 'GFLIB_ControllerPIp_F16', 'horizontalAlignment', 'center');
      | if showStates == 2
      |   color('red');
      |   text(tX,tY - 20, ['debugging mode' char(13) char(10) '(limited performance)'], 'horizontalAlignment', 'center');
      | end
  GFLIB_ControllerPIrAW_F16 : Subsystem  TreatAsAtomicUnit=on  mask(GFLIB_ControllerPIrAW_F16){showStates=Hide (faster execution), resetStatesEnable=Pre-set according to the first set of inputs after reset, f16UpperLimit=0, f16LowerLimit=0, f16CC1sc=0, f16CC2sc=0, u16NShift=0}
      mask prompts: showStates "Show internal states"; resetStatesEnable "Internal state after reset"; f16UpperLimit "f16UpperLimit (Upper Limit of the controller)"; f16LowerLimit "f16LowerLimit (Lower Limit of the controller)"; f16CC1sc "f16CC1sc (CC1 coefficient)"; f16CC2sc "f16CC2sc (CC2 coefficient)"; u16NShift "u16NShift (Scaling bitwise shift applied to the controller coefficients)"
      mask help: Recurrent form PI controller with anti-windup in 16-bit fixed-point fractional implementation. This block supports re-initialization of the internal state during simulation. If the block is reset, the controller's output will be aligned with the input f16ControllerPIrAWOut_preset. Refer to the AMMCLIB User's Guide for further details.
      mask init:
      | if ~evalin('base','exist(''tS8'',''var'')')
      |   if (2 ~= exist('SWLIBS_Typedefs.mat','file'))
      |       error('File SWLIBS_Typedefs.mat is not on the Matlab path. Please add the AMMCLIB "bam" folder in the Matlab Search Path.');
      |   else
      |       evalin('base', 'load(''SWLIBS_Typedefs.mat'')');
      |   end
      | end
      | if showStates == 1
      |     % hidden state variables
      |     if strcmp(get_param([gcb '/f16UpperLimit'], 'BlockType'), 'Inport')
      |         posblk = get_param(gcb, 'Position');
      | 
      |         pos = get_param(    [gcb, '/f16UpperLimit'], 'Position');
      |         orient = get_param( [gcb, '/f16UpperLimit'], 'Orientation');
      |         delete_block(       [gcb, '/f16UpperLimit']);
      |         add_block('built-in/Ground', [gcb, '/f16UpperLimit'], 'Position', pos, 'Orientation', orient);
      | 
      |         pos = get_param(    [gcb, '/f16LowerLimit'], 'Position');
      |         orient = get_param( [gcb, '/f16LowerLimit'], 'Orientation');
      |         delete_block(       [gcb, '/f16LowerLimit']);
      |         add_block('built-in/Ground', [gcb, '/f16LowerLimit'], 'Position', pos, 'Orientation', orient);
      | 
      |         pos = get_param(    [gcb, '/f32Acc'], 'Position');
      |         orient = get_param( [gcb, '/f32Acc'], 'Orientation');
      |         delete_block(       [gcb, '/f32Acc']);
      |         add_block('built-in/Ground', [gcb, '/f32Acc'], 'Position', pos, 'Orientation', orient);
      | 
      |         pos = get_param(    [gcb, '/f16InErrK1'], 'Position');
      |         orient = get_param( [gcb, '/f16InErrK1'], 'Orientation');
      |         delete_block(       [gcb, '/f16InErrK1']);
      |         add_block('built-in/Ground', [gcb, '/f16InErrK1'], 'Position', pos, 'Orientation', orient);
      | 
      |         pos = get_param(    [gcb, '/f16CC1sc'], 'Position');
      |         orient = get_param( [gcb, '/f16CC1sc'], 'Orientation');
      |         delete_block(       [gcb, '/f16CC1sc']);
      |         add_block('built-in/Ground', [gcb, '/f16CC1sc'], 'Position', pos, 'Orientation', orient);
      | 
      |         pos = get_param(    [gcb, '/f16CC2sc'], 'Position');
      |         orient = get_param( [gcb, '/f16CC2sc'], 'Orientation');
      |         delete_block(       [gcb, '/f16CC2sc']);
      |         add_block('built-in/Ground', [gcb, '/f16CC2sc'], 'Position', pos, 'Orientation', orient);
      | 
      |         pos = get_param(    [gcb, '/u16NShift'], 'Position');
      |         orient = get_param( [gcb, '/u16NShift'], 'Orientation');
      |         delete_block(       [gcb, '/u16NShift']);
      |         add_block('built-in/Ground', [gcb, '/u16NShift'], 'Position', pos, 'Orientation', orient);
      | 
      | 
      |         pos = get_param(    [gcb '/f32Acc_Out'], 'Position');
      |         orient = get_param( [gcb '/f32Acc_Out'], 'Orientation');
      |         delete_block(       [gcb '/f32Acc_Out']);
      |         add_block('built-in/Terminator', [gcb '/f32Acc_Out'], 'Position', pos, 'Orientation', orient);
      | 
      |         pos = get_param(    [gcb '/f16InErrK1_Out'], 'Position');
      |         orient = get_param( [gcb '/f16InErrK1_Out'], 'Orientation');
      |         delete_block(       [gcb '/f16InErrK1_Out']);
      |         add_block('built-in/Terminator', [gcb '/f16InErrK1_Out'], 'Position', pos, 'Orientation', orient);
      | 
      | 
      |         set_param([gcb '/f16InErr'], 'Port', '1');
      |         set_param([gcb '/f16ControllerPIrAWOut_preset'], 'Port', '2');
      | 
      |         set_param([gcb '/f16Out'], 'Port', '1');
      | 
      |         set_param(gcb,'MaskEnables',{'on','on','on','on','on','on','on'});
      | 
      |         if (posblk(4) - posblk(2)) > 75
      |           height = 75;
      |           set_param(gcb,'Position',[posblk(1), posblk(2), posblk(3), posblk(2)+height])
      |         end
      |     end
      | else
      |     % shown state variables
      |     if strcmp(get_param([gcb '/f16UpperLimit'], 'BlockType'), 'Ground')
      |         posblk = get_param(gcb, 'Position');
      | 
      |         pos = get_param(    [gcb, '/f16UpperLimit'], 'Position');
      |         orient = get_param( [gcb, '/f16UpperLimit'], 'Orientation');
      |         delete_block(       [gcb, '/f16UpperLimit']);
      |         add_block('built-in/Inport', [gcb, '/f16UpperLimit'], 'Position', pos, 'Orientation', orient, 'OutDataTypeStr', 'int16');
      | 
      |         pos = get_param(    [gcb, '/f16LowerLimit'], 'Position');
      |         orient = get_param( [gcb, '/f16LowerLimit'], 'Orientation');
      |         delete_block(       [gcb, '/f16LowerLimit']);
      |         add_block('built-in/Inport', [gcb, '/f16LowerLimit'], 'Position', pos, 'Orientation', orient, 'OutDataTypeStr', 'int16');
      | 
      |         pos = get_param(    [gcb, '/f32Acc'], 'Position');
      |         orient = get_param( [gcb, '/f32Acc'], 'Orientation');
      |         delete_block(       [gcb, '/f32Acc']);
      |         add_block('built-in/Inport', [gcb, '/f32Acc'], 'Position', pos, 'Orientation', orient, 'OutDataTypeStr', 'int32');
      | 
      |         pos = get_param(    [gcb, '/f16InErrK1'], 'Position');
      |         orient = get_param( [gcb, '/f16InErrK1'], 'Orientation');
      |         delete_block(       [gcb, '/f16InErrK1']);
      |         add_block('built-in/Inport', [gcb, '/f16InErrK1'], 'Position', pos, 'Orientation', orient, 'OutDataTypeStr', 'int16');
      | 
      |         pos = get_param(    [gcb, '/f16CC1sc'], 'Position');
      |         orient = get_param( [gcb, '/f16CC1sc'], 'Orientation');
      |         delete_block(       [gcb, '/f16CC1sc']);
      |         add_block('built-in/Inport', [gcb, '/f16CC1sc'], 'Position', pos, 'Orientation', orient, 'OutDataTypeStr', 'int16');
      | 
      |         pos = get_param(    [gcb, '/f16CC2sc'], 'Position');
      |         orient = get_param( [gcb, '/f16CC2sc'], 'Orientation');
      |         delete_block(       [gcb, '/f16CC2sc']);
      |         add_block('built-in/Inport', [gcb, '/f16CC2sc'], 'Position', pos, 'Orientation', orient, 'OutDataTypeStr', 'int16');
      | 
      |         pos = get_param(    [gcb, '/u16NShift'], 'Position');
      |         orient = get_param( [gcb, '/u16NShift'], 'Orientation');
      |         delete_block(       [gcb, '/u16NShift']);
      |         add_block('built-in/Inport', [gcb, '/u16NShift'], 'Position', pos, 'Orientation', orient, 'OutDataTypeStr', 'uint16');
      | 
      | 
      |         pos = get_param(    [gcb '/f32Acc_Out'], 'Position');
      |         orient = get_param( [gcb '/f32Acc_Out'], 'Orientation');
      |         delete_block(       [gcb '/f32Acc_Out']);
      |         add_block('built-in/Outport', [gcb '/f32Acc_Out'], 'Position', pos, 'Orientation', orient);
      | 
      |         pos = get_param(    [gcb '/f16InErrK1_Out'], 'Position');
      |         orient = get_param( [gcb '/f16InErrK1_Out'], 'Orientation');
      |         delete_block(       [gcb '/f16InErrK1_Out']);
      |         add_block('built-in/Outport', [gcb '/f16InErrK1_Out'], 'Position', pos, 'Orientation', orient);
      | 
      | 
      |         set_param([gcb '/f16InErr'], 'Port', '1');
      |         set_param([gcb '/f16ControllerPIrAWOut_preset'], 'Port', '2');
      |         set_param([gcb '/f16UpperLimit'], 'Port', '3');
      |         set_param([gcb '/f16LowerLimit'], 'Port', '4');
      |         set_param([gcb '/f32Acc'], 'Port', '5');
      |         set_param([gcb '/f16InErrK1'], 'Port', '6');
      |         set_param([gcb '/f16CC1sc'], 'Port', '7');
      |         set_param([gcb '/f16CC2sc'], 'Port', '8');
      |         set_param([gcb '/u16NShift'], 'Port', '9');
      | 
      |         set_param([gcb '/f16Out'], 'Port', '1');
      |         set_param([gcb '/f32Acc_Out'], 'Port', '2');
      |         set_param([gcb '/f16InErrK1_Out'], 'Port', '3');
      | 
      |         set_param(gcb,'MaskEnables',{'on','on','off','off','off','off','off'});
      | 
      |         if (posblk(4) - posblk(2)) < 250
      |           height = 250;
      |           set_param(gcb,'Position',[posblk(1), posblk(2), posblk(3), posblk(2)+height])
      |         end
      |     end
      | end
      settings: RTWSystemCode=Inline
      mask TypeOptions showStates: Hide (faster execution) | Show (allows debugging; connect feedback loops manually)
      mask Callback showStates:
      | maskStr = get_param(gcb,'showStates');
      | if strcmp(maskStr,'Hide (faster execution)'),
      |     set_param(gcb,'MaskEnables',{'on','on','on','on','on','on','on'});
      | else
      |     set_param(gcb,'MaskEnables',{'on','on','off','off','off','off','off'});
      | end
      mask TypeOptions resetStatesEnable: Pre-set according to the first set of inputs after reset | Clear to zero
      mask Display:
      | color('black');
      | pos = get_param(gcb, 'Position');
      | width = pos(3) - pos(1);
      | height = pos(4) - pos(2);
      | tX=width/2;
      | tY=height - 25;
      | color('black');
      | text(tX,tY, 'GFLIB_ControllerPIrAW_F16', 'horizontalAlignment', 'center');
      | if showStates == 2
      |   color('red');
      |   text(tX,tY - 20, ['debugging mode' char(13) char(10) '(limited performance)'], 'horizontalAlignment', 'center');
      | end
  GFLIB_ControllerPIr_F16 : Subsystem  TreatAsAtomicUnit=on  mask(GFLIB_ControllerPIr_F16){showStates=Hide (faster execution), resetStatesEnable=Pre-set according to the first set of inputs after reset, f16CC1=0, f16CC2=0, u16NShift=0}
      mask prompts: showStates "Show internal states"; resetStatesEnable "Internal state after reset"; f16CC1 "f16CC1 (CC1 coefficient)"; f16CC2 "f16CC2 (CC2 coefficient)"; u16NShift "u16NShift (Scaling bitwise shift applied to the controller coefficients)"
      mask help: Reccurent form PI controller without anti-windup in 16-bit fixed-point fractional implementation. This block supports re-initialization of the internal state during simulation. If the block is reset, the controller's output will be aligned with the input f16ControllerPIrOut_preset. Refer to the AMMCLIB User's Guide for further details.
      mask init:
      | if ~evalin('base','exist(''tS8'',''var'')')
      |   if (2 ~= exist('SWLIBS_Typedefs.mat','file'))
      |       error('File SWLIBS_Typedefs.mat is not on the Matlab path. Please add the AMMCLIB "bam" folder in the Matlab Search Path.');
      |   else
      |       evalin('base', 'load(''SWLIBS_Typedefs.mat'')');
      |   end
      | end
      | if showStates == 1
      |     % hidden state variables
      |     if strcmp(get_param([gcb '/f16CC1sc'], 'BlockType'), 'Inport')
      |         posblk = get_param(gcb, 'Position');
      | 
      |         pos = get_param(    [gcb, '/f16CC1sc'], 'Position');
      |         orient = get_param( [gcb, '/f16CC1sc'], 'Orientation');
      |         delete_block(       [gcb, '/f16CC1sc']);
      |         add_block('built-in/Ground', [gcb, '/f16CC1sc'], 'Position', pos, 'Orientation', orient);
      | 
      |         pos = get_param(    [gcb, '/f16CC2sc'], 'Position');
      |         orient = get_param( [gcb, '/f16CC2sc'], 'Orientation');
      |         delete_block(       [gcb, '/f16CC2sc']);
      |         add_block('built-in/Ground', [gcb, '/f16CC2sc'], 'Position', pos, 'Orientation', orient);
      | 
      |         pos = get_param(    [gcb, '/f32Acc'], 'Position');
      |         orient = get_param( [gcb, '/f32Acc'], 'Orientation');
      |         delete_block(       [gcb, '/f32Acc']);
      |         add_block('built-in/Ground', [gcb, '/f32Acc'], 'Position', pos, 'Orientation', orient);
      | 
      |         pos = get_param(    [gcb, '/f16InErrK1'], 'Position');
      |         orient = get_param( [gcb, '/f16InErrK1'], 'Orientation');
      |         delete_block(       [gcb, '/f16InErrK1']);
      |         add_block('built-in/Ground', [gcb, '/f16InErrK1'], 'Position', pos, 'Orientation', orient);
      | 
      |         pos = get_param(    [gcb, '/u16NShift'], 'Position');
      |         orient = get_param( [gcb, '/u16NShift'], 'Orientation');
      |         delete_block(       [gcb, '/u16NShift']);
      |         add_block('built-in/Ground', [gcb, '/u16NShift'], 'Position', pos, 'Orientation', orient);
      | 
      | 
      |         pos = get_param(    [gcb '/f32Acc_Out'], 'Position');
      |         orient = get_param( [gcb '/f32Acc_Out'], 'Orientation');
      |         delete_block(       [gcb '/f32Acc_Out']);
      |         add_block('built-in/Terminator', [gcb '/f32Acc_Out'], 'Position', pos, 'Orientation', orient);
      | 
      |         pos = get_param(    [gcb '/f16InErrK1_Out'], 'Position');
      |         orient = get_param( [gcb '/f16InErrK1_Out'], 'Orientation');
      |         delete_block(       [gcb '/f16InErrK1_Out']);
      |         add_block('built-in/Terminator', [gcb '/f16InErrK1_Out'], 'Position', pos, 'Orientation', orient);
      | 
      | 
      |         set_param([gcb '/f16InErr'], 'Port', '1');
      |         set_param([gcb '/f16ControllerPIrOut_preset'], 'Port', '2');
      | 
      |         set_param([gcb '/f16Out'], 'Port', '1');
      | 
      |         set_param(gcb,'MaskEnables',{'on','on','on','on','on'});
      | 
      |         if (posblk(4) - posblk(2)) > 75
      |           height = 75;
      |           set_param(gcb,'Position',[posblk(1), posblk(2), posblk(3), posblk(2)+height])
      |         end
      |     end
      | else
      |     % shown state variables
      |     if strcmp(get_param([gcb '/f16CC1sc'], 'BlockType'), 'Ground')
      |         posblk = get_param(gcb, 'Position');
      | 
      |         pos = get_param(    [gcb, '/f16CC1sc'], 'Position');
      |         orient = get_param( [gcb, '/f16CC1sc'], 'Orientation');
      |         delete_block(       [gcb, '/f16CC1sc']);
      |         add_block('built-in/Inport', [gcb, '/f16CC1sc'], 'Position', pos, 'Orientation', orient, 'OutDataTypeStr', 'int16');
      | 
      |         pos = get_param(    [gcb, '/f16CC2sc'], 'Position');
      |         orient = get_param( [gcb, '/f16CC2sc'], 'Orientation');
      |         delete_block(       [gcb, '/f16CC2sc']);
      |         add_block('built-in/Inport', [gcb, '/f16CC2sc'], 'Position', pos, 'Orientation', orient, 'OutDataTypeStr', 'int16');
      | 
      |         pos = get_param(    [gcb, '/f32Acc'], 'Position');
      |         orient = get_param( [gcb, '/f32Acc'], 'Orientation');
      |         delete_block(       [gcb, '/f32Acc']);
      |         add_block('built-in/Inport', [gcb, '/f32Acc'], 'Position', pos, 'Orientation', orient, 'OutDataTypeStr', 'int32');
      | 
      |         pos = get_param(    [gcb, '/f16InErrK1'], 'Position');
      |         orient = get_param( [gcb, '/f16InErrK1'], 'Orientation');
      |         delete_block(       [gcb, '/f16InErrK1']);
      |         add_block('built-in/Inport', [gcb, '/f16InErrK1'], 'Position', pos, 'Orientation', orient, 'OutDataTypeStr', 'int16');
      | 
      |         pos = get_param(    [gcb, '/u16NShift'], 'Position');
      |         orient = get_param( [gcb, '/u16NShift'], 'Orientation');
      |         delete_block(       [gcb, '/u16NShift']);
      |         add_block('built-in/Inport', [gcb, '/u16NShift'], 'Position', pos, 'Orientation', orient, 'OutDataTypeStr', 'uint16');
      | 
      | 
      |         pos = get_param(    [gcb '/f32Acc_Out'], 'Position');
      |         orient = get_param( [gcb '/f32Acc_Out'], 'Orientation');
      |         delete_block(       [gcb '/f32Acc_Out']);
      |         add_block('built-in/Outport', [gcb '/f32Acc_Out'], 'Position', pos, 'Orientation', orient);
      | 
      |         pos = get_param(    [gcb '/f16InErrK1_Out'], 'Position');
      |         orient = get_param( [gcb '/f16InErrK1_Out'], 'Orientation');
      |         delete_block(       [gcb '/f16InErrK1_Out']);
      |         add_block('built-in/Outport', [gcb '/f16InErrK1_Out'], 'Position', pos, 'Orientation', orient);
      | 
      | 
      |         set_param([gcb '/f16InErr'], 'Port', '1');
      |         set_param([gcb '/f16ControllerPIrOut_preset'], 'Port', '2');
      |         set_param([gcb '/f16CC1sc'], 'Port', '3');
      |         set_param([gcb '/f16CC2sc'], 'Port', '4');
      |         set_param([gcb '/f32Acc'], 'Port', '5');
      |         set_param([gcb '/f16InErrK1'], 'Port', '6');
      |         set_param([gcb '/u16NShift'], 'Port', '7');
      | 
      |         set_param([gcb '/f16Out'], 'Port', '1');
      |         set_param([gcb '/f32Acc_Out'], 'Port', '2');
      |         set_param([gcb '/f16InErrK1_Out'], 'Port', '3');
      | 
      |         set_param(gcb,'MaskEnables',{'on','on','off','off','off'});
      | 
      |         if (posblk(4) - posblk(2)) < 200
      |           height = 200;
      |           set_param(gcb,'Position',[posblk(1), posblk(2), posblk(3), posblk(2)+height])
      |         end
      |     end
      | end
      settings: RTWSystemCode=Inline
      mask TypeOptions showStates: Hide (faster execution) | Show (allows debugging; connect feedback loops manually)
      mask Callback showStates:
      | maskStr = get_param(gcb,'showStates');
      | if strcmp(maskStr,'Hide (faster execution)'),
      |     set_param(gcb,'MaskEnables',{'on','on','on','on','on'});
      | else
      |     set_param(gcb,'MaskEnables',{'on','on','off','off','off'});
      | end
      mask TypeOptions resetStatesEnable: Pre-set according to the first set of inputs after reset | Clear to zero
      mask Display:
      | color('black');
      | pos = get_param(gcb, 'Position');
      | width = pos(3) - pos(1);
      | height = pos(4) - pos(2);
      | tX=width/2;
      | tY=height - 25;
      | color('black');
      | text(tX,tY, 'GFLIB_ControllerPIr_F16', 'horizontalAlignment', 'center');
      | if showStates == 2
      |   color('red');
      |   text(tX,tY - 20, ['debugging mode' char(13) char(10) '(limited performance)'], 'horizontalAlignment', 'center');
      | end
  GFLIB_Cos_F16 : Subsystem  TreatAsAtomicUnit=on  mask(GFLIB_Cos_F16){}
      mask help: Cosine function in 16-bit fixed-point fractional implementation. Refer to the AMMCLIB User's Guide for further details.
      mask init: same as ammclib_bam/GDFLIB/F16/GDFLIB_FilterFIR_F16
      settings: RTWSystemCode=Inline
      mask Display: pos = get_param(gcb, 'Position');width = pos(3) - pos(1); height = pos(4) - pos(2);tX=width/2;tY=height - 8;color('black');text(tX,tY, 'GFLIB_Cos_F16', 'horizontalAlignment', 'center');
  GFLIB_Hyst_F16 : Subsystem  TreatAsAtomicUnit=on  mask(GFLIB_Hyst_F16){showStates=Hide (faster execution), f16HystOn=0, f16HystOff=0, f16OutValOn=0, f16OutValOff=0}
      mask prompts: showStates "Show internal states"; f16HystOn "f16HystOn (Value determining the upper threshold)"; f16HystOff "f16HystOff (Value determining the lower threshold)"; f16OutValOn "f16OutValOn (Value of the output when input is higher than the upper threshold)"; f16OutValOff "f16OutValOff (Value of the output when input is lower than the lower threshold)"
      mask help: Hysteresis function in 16-bit fixed-point fractional implementation. Refer to the AMMCLIB User's Guide for further details.
      mask init:
      | if ~evalin('base','exist(''tS8'',''var'')')
      |   if (2 ~= exist('SWLIBS_Typedefs.mat','file'))
      |       error('File SWLIBS_Typedefs.mat is not on the Matlab path. Please add the AMMCLIB "bam" folder in the Matlab Search Path.');
      |   else
      |       evalin('base', 'load(''SWLIBS_Typedefs.mat'')');
      |   end
      | end
      | if showStates == 1
      |     % hidden state variables
      |     if strcmp(get_param([gcb '/f16HystOn'], 'BlockType'), 'Inport')
      |         posblk = get_param(gcb, 'Position');
      | 
      |         pos = get_param(    [gcb, '/f16HystOn'], 'Position');
      |         orient = get_param( [gcb, '/f16HystOn'], 'Orientation');
      |         delete_block(       [gcb, '/f16HystOn']);
      |         add_block('built-in/Ground', [gcb, '/f16HystOn'], 'Position', pos, 'Orientation', orient);
      | 
      |         pos = get_param(    [gcb, '/f16HystOff'], 'Position');
      |         orient = get_param( [gcb, '/f16HystOff'], 'Orientation');
      |         delete_block(       [gcb, '/f16HystOff']);
      |         add_block('built-in/Ground', [gcb, '/f16HystOff'], 'Position', pos, 'Orientation', orient);
      | 
      |         pos = get_param(    [gcb, '/f16OutValOn'], 'Position');
      |         orient = get_param( [gcb, '/f16OutValOn'], 'Orientation');
      |         delete_block(       [gcb, '/f16OutValOn']);
      |         add_block('built-in/Ground', [gcb, '/f16OutValOn'], 'Position', pos, 'Orientation', orient);
      | 
      |         pos = get_param(    [gcb, '/f16OutValOff'], 'Position');
      |         orient = get_param( [gcb, '/f16OutValOff'], 'Orientation');
      |         delete_block(       [gcb, '/f16OutValOff']);
      |         add_block('built-in/Ground', [gcb, '/f16OutValOff'], 'Position', pos, 'Orientation', orient);
      | 
      |         pos = get_param(    [gcb, '/f16OutState'], 'Position');
      |         orient = get_param( [gcb, '/f16OutState'], 'Orientation');
      |         delete_block(       [gcb, '/f16OutState']);
      |         add_block('built-in/Ground', [gcb, '/f16OutState'], 'Position', pos, 'Orientation', orient);
      | 
      | 
      |         pos = get_param(    [gcb '/f16OutState_Out'], 'Position');
      |         orient = get_param( [gcb '/f16OutState_Out'], 'Orientation');
      |         delete_block(       [gcb '/f16OutState_Out']);
      |         add_block('built-in/Terminator', [gcb '/f16OutState_Out'], 'Position', pos, 'Orientation', orient);
      | 
      | 
      |         set_param([gcb '/f16In'], 'Port', '1');
      | 
      |         set_param([gcb '/f16Out'], 'Port', '1');
      | 
      |         set_param(gcb,'MaskEnables',{'on','on','on','on','on'});
      | 
      |         if (posblk(4) - posblk(2)) > 50
      |           height = 50;
      |           set_param(gcb,'Position',[posblk(1), posblk(2), posblk(3), posblk(2)+height])
      |         end
      |     end
      | else
      |     % shown state variables
      |     if strcmp(get_param([gcb '/f16HystOn'], 'BlockType'), 'Ground')
      |         posblk = get_param(gcb, 'Position');
      | 
      |         pos = get_param(    [gcb, '/f16HystOn'], 'Position');
      |         orient = get_param( [gcb, '/f16HystOn'], 'Orientation');
      |         delete_block(       [gcb, '/f16HystOn']);
      |         add_block('built-in/Inport', [gcb, '/f16HystOn'], 'Position', pos, 'Orientation', orient, 'OutDataTypeStr', 'int16');
      | 
      |         pos = get_param(    [gcb, '/f16HystOff'], 'Position');
      |         orient = get_param( [gcb, '/f16HystOff'], 'Orientation');
      |         delete_block(       [gcb, '/f16HystOff']);
      |         add_block('built-in/Inport', [gcb, '/f16HystOff'], 'Position', pos, 'Orientation', orient, 'OutDataTypeStr', 'int16');
      | 
      |         pos = get_param(    [gcb, '/f16OutValOn'], 'Position');
      |         orient = get_param( [gcb, '/f16OutValOn'], 'Orientation');
      |         delete_block(       [gcb, '/f16OutValOn']);
      |         add_block('built-in/Inport', [gcb, '/f16OutValOn'], 'Position', pos, 'Orientation', orient, 'OutDataTypeStr', 'int16');
      | 
      |         pos = get_param(    [gcb, '/f16OutValOff'], 'Position');
      |         orient = get_param( [gcb, '/f16OutValOff'], 'Orientation');
      |         delete_block(       [gcb, '/f16OutValOff']);
      |         add_block('built-in/Inport', [gcb, '/f16OutValOff'], 'Position', pos, 'Orientation', orient, 'OutDataTypeStr', 'int16');
      | 
      |         pos = get_param(    [gcb, '/f16OutState'], 'Position');
      |         orient = get_param( [gcb, '/f16OutState'], 'Orientation');
      |         delete_block(       [gcb, '/f16OutState']);
      |         add_block('built-in/Inport', [gcb, '/f16OutState'], 'Position', pos, 'Orientation', orient, 'OutDataTypeStr', 'int16');
      | 
      | 
      |         pos = get_param(    [gcb '/f16OutState_Out'], 'Position');
      |         orient = get_param( [gcb '/f16OutState_Out'], 'Orientation');
      |         delete_block(       [gcb '/f16OutState_Out']);
      |         add_block('built-in/Outport', [gcb '/f16OutState_Out'], 'Position', pos, 'Orientation', orient);
      | 
      | 
      |         set_param([gcb '/f16In'], 'Port', '1');
      |         set_param([gcb '/f16HystOn'], 'Port', '2');
      |         set_param([gcb '/f16HystOff'], 'Port', '3');
      |         set_param([gcb '/f16OutValOn'], 'Port', '4');
      |         set_param([gcb '/f16OutValOff'], 'Port', '5');
      |         set_param([gcb '/f16OutState'], 'Port', '6');
      | 
      |         set_param([gcb '/f16Out'], 'Port', '1');
      |         set_param([gcb '/f16OutState_Out'], 'Port', '2');
      | 
      |         set_param(gcb,'MaskEnables',{'on','off','off','off','off'});
      | 
      |         if (posblk(4) - posblk(2)) < 175
      |           height = 175;
      |           set_param(gcb,'Position',[posblk(1), posblk(2), posblk(3), posblk(2)+height])
      |         end
      |     end
      | end
      settings: RTWSystemCode=Inline
      mask TypeOptions showStates: Hide (faster execution) | Show (allows debugging; connect feedback loops manually)
      mask Callback showStates:
      | maskStr = get_param(gcb,'showStates');
      | if strcmp(maskStr,'Hide (faster execution)'),
      |     set_param(gcb,'MaskEnables',{'on','on','on','on','on'});
      | else
      |     set_param(gcb,'MaskEnables',{'on','off','off','off','off'});
      | end
      mask Display:
      | color('black');
      | pos = get_param(gcb, 'Position');
      | width = pos(3) - pos(1);
      | height = pos(4) - pos(2);
      | tX=width/2;
      | tY=height - 8;
      | color('black');
      | text(tX,tY, 'GFLIB_Hyst_F16', 'horizontalAlignment', 'center');
      | if showStates == 2
      |   color('red');
      |   text(tX,tY - 20, ['debugging mode' char(13) char(10) '(limited performance)'], 'horizontalAlignment', 'center');
      | end
  GFLIB_IntegratorTR_F16 : Subsystem  TreatAsAtomicUnit=on  mask(GFLIB_IntegratorTR_F16){showStates=Hide (faster execution), resetStatesEnable=Pre-set according to the first set of inputs after reset, f16C1=0, u16NShift=0}
      mask prompts: showStates "Show internal states"; resetStatesEnable "Internal state after reset"; f16C1 "f16C1 (Integrator coefficient)"; u16NShift "u16NShift (Scaling bitwise shift applied to the integrator coefficient)"
      mask help: Discrete integrator transformed from a linear model using Billinear (trapezoidal) transformation in 16-bit fixed-point fractional implementation. This block supports re-initialization of the internal state during simulation. If the block is reset, the integrator's output will be aligned with the input f16IntegratorTROut_preset. Refer to the AMMCLIB User's Guide for further details.
      mask init:
      | if ~evalin('base','exist(''tS8'',''var'')')
      |   if (2 ~= exist('SWLIBS_Typedefs.mat','file'))
      |       error('File SWLIBS_Typedefs.mat is not on the Matlab path. Please add the AMMCLIB "bam" folder in the Matlab Search Path.');
      |   else
      |       evalin('base', 'load(''SWLIBS_Typedefs.mat'')');
      |   end
      | end
      | if showStates == 1
      |     % hidden state variables
      |     if strcmp(get_param([gcb '/f16C1'], 'BlockType'), 'Inport')
      |         posblk = get_param(gcb, 'Position');
      | 
      |         pos = get_param(    [gcb, '/f16C1'], 'Position');
      |         orient = get_param( [gcb, '/f16C1'], 'Orientation');
      |         delete_block(       [gcb, '/f16C1']);
      |         add_block('built-in/Ground', [gcb, '/f16C1'], 'Position', pos, 'Orientation', orient);
      | 
      |         pos = get_param(    [gcb, '/u16NShift'], 'Position');
      |         orient = get_param( [gcb, '/u16NShift'], 'Orientation');
      |         delete_block(       [gcb, '/u16NShift']);
      |         add_block('built-in/Ground', [gcb, '/u16NShift'], 'Position', pos, 'Orientation', orient);
      | 
      |         pos = get_param(    [gcb, '/f32State'], 'Position');
      |         orient = get_param( [gcb, '/f32State'], 'Orientation');
      |         delete_block(       [gcb, '/f32State']);
      |         add_block('built-in/Ground', [gcb, '/f32State'], 'Position', pos, 'Orientation', orient);
      | 
      |         pos = get_param(    [gcb, '/f16InK1'], 'Position');
      |         orient = get_param( [gcb, '/f16InK1'], 'Orientation');
      |         delete_block(       [gcb, '/f16InK1']);
      |         add_block('built-in/Ground', [gcb, '/f16InK1'], 'Position', pos, 'Orientation', orient);
      | 
      | 
      |         pos = get_param(    [gcb '/f32State_Out'], 'Position');
      |         orient = get_param( [gcb '/f32State_Out'], 'Orientation');
      |         delete_block(       [gcb '/f32State_Out']);
      |         add_block('built-in/Terminator', [gcb '/f32State_Out'], 'Position', pos, 'Orientation', orient);
      | 
      |         pos = get_param(    [gcb '/f16InK1_Out'], 'Position');
      |         orient = get_param( [gcb '/f16InK1_Out'], 'Orientation');
      |         delete_block(       [gcb '/f16InK1_Out']);
      |         add_block('built-in/Terminator', [gcb '/f16InK1_Out'], 'Position', pos, 'Orientation', orient);
      | 
      | 
      |         set_param([gcb '/f16In'], 'Port', '1');
      |         set_param([gcb '/f16IntegratorTROut_preset'], 'Port', '2');
      | 
      |         set_param([gcb '/f16Out'], 'Port', '1');
      | 
      |         set_param(gcb,'MaskEnables',{'on','on','on','on'});
      | 
      |         if (posblk(4) - posblk(2)) > 75
      |           height = 75;
      |           set_param(gcb,'Position',[posblk(1), posblk(2), posblk(3), posblk(2)+height])
      |         end
      |     end
      | else
      |     % shown state variables
      |     if strcmp(get_param([gcb '/f16C1'], 'BlockType'), 'Ground')
      |         posblk = get_param(gcb, 'Position');
      | 
      |         pos = get_param(    [gcb, '/f16C1'], 'Position');
      |         orient = get_param( [gcb, '/f16C1'], 'Orientation');
      |         delete_block(       [gcb, '/f16C1']);
      |         add_block('built-in/Inport', [gcb, '/f16C1'], 'Position', pos, 'Orientation', orient, 'OutDataTypeStr', 'int16');
      | 
      |         pos = get_param(    [gcb, '/u16NShift'], 'Position');
      |         orient = get_param( [gcb, '/u16NShift'], 'Orientation');
      |         delete_block(       [gcb, '/u16NShift']);
      |         add_block('built-in/Inport', [gcb, '/u16NShift'], 'Position', pos, 'Orientation', orient, 'OutDataTypeStr', 'uint16');
      | 
      |         pos = get_param(    [gcb, '/f32State'], 'Position');
      |         orient = get_param( [gcb, '/f32State'], 'Orientation');
      |         delete_block(       [gcb, '/f32State']);
      |         add_block('built-in/Inport', [gcb, '/f32State'], 'Position', pos, 'Orientation', orient, 'OutDataTypeStr', 'int32');
      | 
      |         pos = get_param(    [gcb, '/f16InK1'], 'Position');
      |         orient = get_param( [gcb, '/f16InK1'], 'Orientation');
      |         delete_block(       [gcb, '/f16InK1']);
      |         add_block('built-in/Inport', [gcb, '/f16InK1'], 'Position', pos, 'Orientation', orient, 'OutDataTypeStr', 'int16');
      | 
      | 
      |         pos = get_param(    [gcb '/f32State_Out'], 'Position');
      |         orient = get_param( [gcb '/f32State_Out'], 'Orientation');
      |         delete_block(       [gcb '/f32State_Out']);
      |         add_block('built-in/Outport', [gcb '/f32State_Out'], 'Position', pos, 'Orientation', orient);
      | 
      |         pos = get_param(    [gcb '/f16InK1_Out'], 'Position');
      |         orient = get_param( [gcb '/f16InK1_Out'], 'Orientation');
      |         delete_block(       [gcb '/f16InK1_Out']);
      |         add_block('built-in/Outport', [gcb '/f16InK1_Out'], 'Position', pos, 'Orientation', orient);
      | 
      | 
      |         set_param([gcb '/f16In'], 'Port', '1');
      |         set_param([gcb '/f16IntegratorTROut_preset'], 'Port', '2');
      |         set_param([gcb '/f16C1'], 'Port', '3');
      |         set_param([gcb '/u16NShift'], 'Port', '4');
      |         set_param([gcb '/f32State'], 'Port', '5');
      |         set_param([gcb '/f16InK1'], 'Port', '6');
      | 
      |         set_param([gcb '/f16Out'], 'Port', '1');
      |         set_param([gcb '/f32State_Out'], 'Port', '2');
      |         set_param([gcb '/f16InK1_Out'], 'Port', '3');
      | 
      |         set_param(gcb,'MaskEnables',{'on','on','off','off'});
      | 
      |         if (posblk(4) - posblk(2)) < 175
      |           height = 175;
      |           set_param(gcb,'Position',[posblk(1), posblk(2), posblk(3), posblk(2)+height])
      |         end
      |     end
      | end
      settings: RTWSystemCode=Inline
      mask TypeOptions showStates: Hide (faster execution) | Show (allows debugging; connect feedback loops manually)
      mask Callback showStates:
      | maskStr = get_param(gcb,'showStates');
      | if strcmp(maskStr,'Hide (faster execution)'),
      |     set_param(gcb,'MaskEnables',{'on','on','on','on'});
      | else
      |     set_param(gcb,'MaskEnables',{'on','on','off','off'});
      | end
      mask TypeOptions resetStatesEnable: Pre-set according to the first set of inputs after reset | Clear to zero
      mask Display:
      | color('black');
      | pos = get_param(gcb, 'Position');
      | width = pos(3) - pos(1);
      | height = pos(4) - pos(2);
      | tX=width/2;
      | tY=height - 25;
      | color('black');
      | text(tX,tY, 'GFLIB_IntegratorTR_F16', 'horizontalAlignment', 'center');
      | if showStates == 2
      |   color('red');
      |   text(tX,tY - 20, ['debugging mode' char(13) char(10) '(limited performance)'], 'horizontalAlignment', 'center');
      | end
  GFLIB_Limit_F16 : Subsystem  TreatAsAtomicUnit=on  mask(GFLIB_Limit_F16){showStates=Hide (faster execution), f16LowerLimit=0, f16UpperLimit=0}
      mask prompts: showStates "Show internal states"; f16LowerLimit "f16LowerLimit (Lower limit)"; f16UpperLimit "f16UpperLimit (Upper limit)"
      mask help: Limit function in 16-bit fixed-point fractional implementation. Refer to the AMMCLIB User's Guide for further details.
      mask init:
      | if ~evalin('base','exist(''tS8'',''var'')')
      |   if (2 ~= exist('SWLIBS_Typedefs.mat','file'))
      |       error('File SWLIBS_Typedefs.mat is not on the Matlab path. Please add the AMMCLIB "bam" folder in the Matlab Search Path.');
      |   else
      |       evalin('base', 'load(''SWLIBS_Typedefs.mat'')');
      |   end
      | end
      | if showStates == 1
      |     % hidden state variables
      |     if strcmp(get_param([gcb '/f16LowerLimit'], 'BlockType'), 'Inport')
      |         posblk = get_param(gcb, 'Position');
      | 
      |         pos = get_param(    [gcb, '/f16LowerLimit'], 'Position');
      |         orient = get_param( [gcb, '/f16LowerLimit'], 'Orientation');
      |         delete_block(       [gcb, '/f16LowerLimit']);
      |         add_block('built-in/Ground', [gcb, '/f16LowerLimit'], 'Position', pos, 'Orientation', orient);
      | 
      |         pos = get_param(    [gcb, '/f16UpperLimit'], 'Position');
      |         orient = get_param( [gcb, '/f16UpperLimit'], 'Orientation');
      |         delete_block(       [gcb, '/f16UpperLimit']);
      |         add_block('built-in/Ground', [gcb, '/f16UpperLimit'], 'Position', pos, 'Orientation', orient);
      | 
      | 
      | 
      |         set_param([gcb '/f16In'], 'Port', '1');
      | 
      |         set_param([gcb '/f16Out'], 'Port', '1');
      | 
      |         set_param(gcb,'MaskEnables',{'on','on','on'});
      | 
      |         if (posblk(4) - posblk(2)) > 50
      |           height = 50;
      |           set_param(gcb,'Position',[posblk(1), posblk(2), posblk(3), posblk(2)+height])
      |         end
      |     end
      | else
      |     % shown state variables
      |     if strcmp(get_param([gcb '/f16LowerLimit'], 'BlockType'), 'Ground')
      |         posblk = get_param(gcb, 'Position');
      | 
      |         pos = get_param(    [gcb, '/f16LowerLimit'], 'Position');
      |         orient = get_param( [gcb, '/f16LowerLimit'], 'Orientation');
      |         delete_block(       [gcb, '/f16LowerLimit']);
      |         add_block('built-in/Inport', [gcb, '/f16LowerLimit'], 'Position', pos, 'Orientation', orient, 'OutDataTypeStr', 'int16');
      | 
      |         pos = get_param(    [gcb, '/f16UpperLimit'], 'Position');
      |         orient = get_param( [gcb, '/f16UpperLimit'], 'Orientation');
      |         delete_block(       [gcb, '/f16UpperLimit']);
      |         add_block('built-in/Inport', [gcb, '/f16UpperLimit'], 'Position', pos, 'Orientation', orient, 'OutDataTypeStr', 'int16');
      | 
      | 
      | 
      |         set_param([gcb '/f16In'], 'Port', '1');
      |         set_param([gcb '/f16LowerLimit'], 'Port', '2');
      |         set_param([gcb '/f16UpperLimit'], 'Port', '3');
      | 
      |         set_param([gcb '/f16Out'], 'Port', '1');
      | 
      |         set_param(gcb,'MaskEnables',{'on','off','off'});
      | 
      |         if (posblk(4) - posblk(2)) < 100
      |           height = 100;
      |           set_param(gcb,'Position',[posblk(1), posblk(2), posblk(3), posblk(2)+height])
      |         end
      |     end
      | end
      settings: RTWSystemCode=Inline
      mask TypeOptions showStates: Hide (faster execution) | Show (allows debugging; connect feedback loops manually)
      mask Callback showStates:
      | maskStr = get_param(gcb,'showStates');
      | if strcmp(maskStr,'Hide (faster execution)'),
      |     set_param(gcb,'MaskEnables',{'on','on','on'});
      | else
      |     set_param(gcb,'MaskEnables',{'on','off','off'});
      | end
      mask Display:
      | color('black');
      | pos = get_param(gcb, 'Position');
      | width = pos(3) - pos(1);
      | height = pos(4) - pos(2);
      | tX=width/2;
      | tY=height - 8;
      | color('black');
      | text(tX,tY, 'GFLIB_Limit_F16', 'horizontalAlignment', 'center');
      | if showStates == 2
      |   color('red');
      |   text(tX,tY - 20, ['debugging mode' char(13) char(10) '(limited performance)'], 'horizontalAlignment', 'center');
      | end
  GFLIB_LowerLimit_F16 : Subsystem  TreatAsAtomicUnit=on  mask(GFLIB_LowerLimit_F16){showStates=Hide (faster execution), f16LowerLimit=0}
      mask prompts: showStates "Show internal states"; f16LowerLimit "f16LowerLimit (Value determining the lower limit threshold)"
      mask help: Lower limit function in 16-bit fixed-point fractional implementation. Refer to the AMMCLIB User's Guide for further details.
      mask init:
      | if ~evalin('base','exist(''tS8'',''var'')')
      |   if (2 ~= exist('SWLIBS_Typedefs.mat','file'))
      |       error('File SWLIBS_Typedefs.mat is not on the Matlab path. Please add the AMMCLIB "bam" folder in the Matlab Search Path.');
      |   else
      |       evalin('base', 'load(''SWLIBS_Typedefs.mat'')');
      |   end
      | end
      | if showStates == 1
      |     % hidden state variables
      |     if strcmp(get_param([gcb '/f16LowerLimit'], 'BlockType'), 'Inport')
      |         posblk = get_param(gcb, 'Position');
      | 
      |         pos = get_param(    [gcb, '/f16LowerLimit'], 'Position');
      |         orient = get_param( [gcb, '/f16LowerLimit'], 'Orientation');
      |         delete_block(       [gcb, '/f16LowerLimit']);
      |         add_block('built-in/Ground', [gcb, '/f16LowerLimit'], 'Position', pos, 'Orientation', orient);
      | 
      | 
      | 
      |         set_param([gcb '/f16In'], 'Port', '1');
      | 
      |         set_param([gcb '/f16Out'], 'Port', '1');
      | 
      |         set_param(gcb,'MaskEnables',{'on','on'});
      | 
      |         if (posblk(4) - posblk(2)) > 50
      |           height = 50;
      |           set_param(gcb,'Position',[posblk(1), posblk(2), posblk(3), posblk(2)+height])
      |         end
      |     end
      | else
      |     % shown state variables
      |     if strcmp(get_param([gcb '/f16LowerLimit'], 'BlockType'), 'Ground')
      |         posblk = get_param(gcb, 'Position');
      | 
      |         pos = get_param(    [gcb, '/f16LowerLimit'], 'Position');
      |         orient = get_param( [gcb, '/f16LowerLimit'], 'Orientation');
      |         delete_block(       [gcb, '/f16LowerLimit']);
      |         add_block('built-in/Inport', [gcb, '/f16LowerLimit'], 'Position', pos, 'Orientation', orient, 'OutDataTypeStr', 'int16');
      | 
      | 
      | 
      |         set_param([gcb '/f16In'], 'Port', '1');
      |         set_param([gcb '/f16LowerLimit'], 'Port', '2');
      | 
      |         set_param([gcb '/f16Out'], 'Port', '1');
      | 
      |         set_param(gcb,'MaskEnables',{'on','off'});
      | 
      |         if (posblk(4) - posblk(2)) < 75
      |           height = 75;
      |           set_param(gcb,'Position',[posblk(1), posblk(2), posblk(3), posblk(2)+height])
      |         end
      |     end
      | end
      settings: RTWSystemCode=Inline
      mask TypeOptions showStates: Hide (faster execution) | Show (allows debugging; connect feedback loops manually)
      mask Callback showStates:
      | maskStr = get_param(gcb,'showStates');
      | if strcmp(maskStr,'Hide (faster execution)'),
      |     set_param(gcb,'MaskEnables',{'on','on'});
      | else
      |     set_param(gcb,'MaskEnables',{'on','off'});
      | end
      mask Display:
      | color('black');
      | pos = get_param(gcb, 'Position');
      | width = pos(3) - pos(1);
      | height = pos(4) - pos(2);
      | tX=width/2;
      | tY=height - 8;
      | color('black');
      | text(tX,tY, 'GFLIB_LowerLimit_F16', 'horizontalAlignment', 'center');
      | if showStates == 2
      |   color('red');
      |   text(tX,tY - 20, ['debugging mode' char(13) char(10) '(limited performance)'], 'horizontalAlignment', 'center');
      | end
  GFLIB_Lut1D_F16 : Subsystem  TreatAsAtomicUnit=on  mask(GFLIB_Lut1D_F16){pf16Table=2^15*[-0.75 -0.25 0.0 0.25 0.75], s16MidIdx=2}
      mask prompts: pf16Table "pf16Table (Vector holding the ordinate values of interpolating intervals)"; s16MidIdx "Middle index in the table pf16Table (zero-based indexing)"
      mask help: One dimensional lookup table function in 16-bit fixed-point fractional implementation. Refer to the AMMCLIB User's Guide for further details.
      mask init: same as ammclib_bam/GDFLIB/F16/GDFLIB_FilterFIR_F16
      settings: RTWSystemCode=Inline
      mask Display: pos = get_param(gcb, 'Position');width = pos(3) - pos(1); height = pos(4) - pos(2);tX=width/2;tY=height - 8;color('black');text(tX,tY, 'GFLIB_Lut1D_F16', 'horizontalAlignment', 'center');
  GFLIB_Lut2D_F16 : Subsystem  TreatAsAtomicUnit=on  mask(GFLIB_Lut2D_F16){pf16Table=2^15*[-0.75 0.0 0.75; -0.5 0.0 0.5; -0.25 0.0 0.25], s16MidIdx=4}
      mask prompts: pf16Table "pf16Table (Matrix of z-coordinate values at vertices)"; s16MidIdx "Middle index in the table pf16Table (zero-based indexing over all elements)"
      mask help: Two dimensional lookup table function in 16-bit fixed-point fractional implementation. Refer to the AMMCLIB User's Guide for further details.
      mask init: same as ammclib_bam/GDFLIB/F16/GDFLIB_FilterFIR_F16
      settings: RTWSystemCode=Inline
      mask Display: pos = get_param(gcb, 'Position');width = pos(3) - pos(1); height = pos(4) - pos(2);tX=width/2;tY=height - 8;color('black');text(tX,tY, 'GFLIB_Lut2D_F16', 'horizontalAlignment', 'center');
  GFLIB_Ramp_F16 : Subsystem  TreatAsAtomicUnit=on  mask(GFLIB_Ramp_F16){showStates=Hide (faster execution), f16RampUp=0, f16RampDown=0}
      mask prompts: showStates "Show internal states"; f16RampUp "f16RampUp (Ramp up increment coefficient)"; f16RampDown "f16RampDown (Ramp decrement coefficient)"
      mask help: Rate of change limiter - ramp function in 16-bit fixed-point fractional implementation. Refer to the AMMCLIB User's Guide for further details.
      mask init:
      | if ~evalin('base','exist(''tS8'',''var'')')
      |   if (2 ~= exist('SWLIBS_Typedefs.mat','file'))
      |       error('File SWLIBS_Typedefs.mat is not on the Matlab path. Please add the AMMCLIB "bam" folder in the Matlab Search Path.');
      |   else
      |       evalin('base', 'load(''SWLIBS_Typedefs.mat'')');
      |   end
      | end
      | if showStates == 1
      |     % hidden state variables
      |     if strcmp(get_param([gcb '/f16State'], 'BlockType'), 'Inport')
      |         posblk = get_param(gcb, 'Position');
      | 
      |         pos = get_param(    [gcb, '/f16State'], 'Position');
      |         orient = get_param( [gcb, '/f16State'], 'Orientation');
      |         delete_block(       [gcb, '/f16State']);
      |         add_block('built-in/Ground', [gcb, '/f16State'], 'Position', pos, 'Orientation', orient);
      | 
      |         pos = get_param(    [gcb, '/f16RampUp'], 'Position');
      |         orient = get_param( [gcb, '/f16RampUp'], 'Orientation');
      |         delete_block(       [gcb, '/f16RampUp']);
      |         add_block('built-in/Ground', [gcb, '/f16RampUp'], 'Position', pos, 'Orientation', orient);
      | 
      |         pos = get_param(    [gcb, '/f16RampDown'], 'Position');
      |         orient = get_param( [gcb, '/f16RampDown'], 'Orientation');
      |         delete_block(       [gcb, '/f16RampDown']);
      |         add_block('built-in/Ground', [gcb, '/f16RampDown'], 'Position', pos, 'Orientation', orient);
      | 
      | 
      |         pos = get_param(    [gcb '/f16State_Out'], 'Position');
      |         orient = get_param( [gcb '/f16State_Out'], 'Orientation');
      |         delete_block(       [gcb '/f16State_Out']);
      |         add_block('built-in/Terminator', [gcb '/f16State_Out'], 'Position', pos, 'Orientation', orient);
      | 
      | 
      |         set_param([gcb '/f16In'], 'Port', '1');
      | 
      |         set_param([gcb '/f16Out'], 'Port', '1');
      | 
      |         set_param(gcb,'MaskEnables',{'on','on','on'});
      | 
      |         if (posblk(4) - posblk(2)) > 50
      |           height = 50;
      |           set_param(gcb,'Position',[posblk(1), posblk(2), posblk(3), posblk(2)+height])
      |         end
      |     end
      | else
      |     % shown state variables
      |     if strcmp(get_param([gcb '/f16State'], 'BlockType'), 'Ground')
      |         posblk = get_param(gcb, 'Position');
      | 
      |         pos = get_param(    [gcb, '/f16State'], 'Position');
      |         orient = get_param( [gcb, '/f16State'], 'Orientation');
      |         delete_block(       [gcb, '/f16State']);
      |         add_block('built-in/Inport', [gcb, '/f16State'], 'Position', pos, 'Orientation', orient, 'OutDataTypeStr', 'int16');
      | 
      |         pos = get_param(    [gcb, '/f16RampUp'], 'Position');
      |         orient = get_param( [gcb, '/f16RampUp'], 'Orientation');
      |         delete_block(       [gcb, '/f16RampUp']);
      |         add_block('built-in/Inport', [gcb, '/f16RampUp'], 'Position', pos, 'Orientation', orient, 'OutDataTypeStr', 'int16');
      | 
      |         pos = get_param(    [gcb, '/f16RampDown'], 'Position');
      |         orient = get_param( [gcb, '/f16RampDown'], 'Orientation');
      |         delete_block(       [gcb, '/f16RampDown']);
      |         add_block('built-in/Inport', [gcb, '/f16RampDown'], 'Position', pos, 'Orientation', orient, 'OutDataTypeStr', 'int16');
      | 
      | 
      |         pos = get_param(    [gcb '/f16State_Out'], 'Position');
      |         orient = get_param( [gcb '/f16State_Out'], 'Orientation');
      |         delete_block(       [gcb '/f16State_Out']);
      |         add_block('built-in/Outport', [gcb '/f16State_Out'], 'Position', pos, 'Orientation', orient);
      | 
      | 
      |         set_param([gcb '/f16In'], 'Port', '1');
      |         set_param([gcb '/f16State'], 'Port', '2');
      |         set_param([gcb '/f16RampUp'], 'Port', '3');
      |         set_param([gcb '/f16RampDown'], 'Port', '4');
      | 
      |         set_param([gcb '/f16Out'], 'Port', '1');
      |         set_param([gcb '/f16State_Out'], 'Port', '2');
      | 
      |         set_param(gcb,'MaskEnables',{'on','off','off'});
      | 
      |         if (posblk(4) - posblk(2)) < 125
      |           height = 125;
      |           set_param(gcb,'Position',[posblk(1), posblk(2), posblk(3), posblk(2)+height])
      |         end
      |     end
      | end
      settings: RTWSystemCode=Inline
      mask TypeOptions showStates: Hide (faster execution) | Show (allows debugging; connect feedback loops manually)
      mask Callback showStates:
      | maskStr = get_param(gcb,'showStates');
      | if strcmp(maskStr,'Hide (faster execution)'),
      |     set_param(gcb,'MaskEnables',{'on','on','on'});
      | else
      |     set_param(gcb,'MaskEnables',{'on','off','off'});
      | end
      mask Display:
      | color('black');
      | pos = get_param(gcb, 'Position');
      | width = pos(3) - pos(1);
      | height = pos(4) - pos(2);
      | tX=width/2;
      | tY=height - 8;
      | color('black');
      | text(tX,tY, 'GFLIB_Ramp_F16', 'horizontalAlignment', 'center');
      | if showStates == 2
      |   color('red');
      |   text(tX,tY - 20, ['debugging mode' char(13) char(10) '(limited performance)'], 'horizontalAlignment', 'center');
      | end
  GFLIB_Sign_F16 : Subsystem  TreatAsAtomicUnit=on  mask(GFLIB_Sign_F16){}
      mask help: Bit accurate model of GFLIB_Sign function in 16-bit fixed-point fractional implementation. Refer to the AMMCLIB User's Guide for further details.
      mask init: same as ammclib_bam/GDFLIB/F16/GDFLIB_FilterFIR_F16
      settings: RTWSystemCode=Inline
      mask Display: pos = get_param(gcb, 'Position');width = pos(3) - pos(1); height = pos(4) - pos(2);tX=width/2;tY=height - 8;color('black');text(tX,tY, 'GFLIB_Sign_F16', 'horizontalAlignment', 'center');
  GFLIB_SinCos_F16 : Subsystem  TreatAsAtomicUnit=on  mask(GFLIB_SinCos_F16){}
      mask help: Calculation of sine and cosine of the same argument in 16-bit fixed-point fractional implementation. Refer to the AMMCLIB User's Guide for further details.
      mask init: same as ammclib_bam/GDFLIB/F16/GDFLIB_FilterFIR_F16
      settings: RTWSystemCode=Inline
      mask Display: pos = get_param(gcb, 'Position');width = pos(3) - pos(1); height = pos(4) - pos(2);tX=width/2;tY=height - 8;color('black');text(tX,tY, 'GFLIB_SinCos_F16', 'horizontalAlignment', 'center');
  GFLIB_Sin_F16 : Subsystem  TreatAsAtomicUnit=on  mask(GFLIB_Sin_F16){}
      mask help: Sine function in 16-bit fixed-point fractional implementation. Refer to the AMMCLIB User's Guide for further details.
      mask init: same as ammclib_bam/GDFLIB/F16/GDFLIB_FilterFIR_F16
      settings: RTWSystemCode=Inline
      mask Display: pos = get_param(gcb, 'Position');width = pos(3) - pos(1); height = pos(4) - pos(2);tX=width/2;tY=height - 8;color('black');text(tX,tY, 'GFLIB_Sin_F16', 'horizontalAlignment', 'center');
  GFLIB_Sqrt_F16 : Subsystem  TreatAsAtomicUnit=on  mask(GFLIB_Sqrt_F16){}
      mask help: Square root approximation in 16-bit fixed-point fractional implementation. Refer to the AMMCLIB User's Guide for further details.
      mask init: same as ammclib_bam/GDFLIB/F16/GDFLIB_FilterFIR_F16
      settings: RTWSystemCode=Inline
      mask Display: pos = get_param(gcb, 'Position');width = pos(3) - pos(1); height = pos(4) - pos(2);tX=width/2;tY=height - 8;color('black');text(tX,tY, 'GFLIB_Sqrt_F16', 'horizontalAlignment', 'center');
  GFLIB_Tan_F16 : Subsystem  TreatAsAtomicUnit=on  mask(GFLIB_Tan_F16){}
      mask help: Tangent function in 16-bit fixed-point fractional implementation. Refer to the AMMCLIB User's Guide for further details.
      mask init: same as ammclib_bam/GDFLIB/F16/GDFLIB_FilterFIR_F16
      settings: RTWSystemCode=Inline
      mask Display: pos = get_param(gcb, 'Position');width = pos(3) - pos(1); height = pos(4) - pos(2);tX=width/2;tY=height - 8;color('black');text(tX,tY, 'GFLIB_Tan_F16', 'horizontalAlignment', 'center');
  GFLIB_UpperLimit_F16 : Subsystem  TreatAsAtomicUnit=on  mask(GFLIB_UpperLimit_F16){showStates=Hide (faster execution), f16UpperLimit=0}
      mask prompts: showStates "Show internal states"; f16UpperLimit "f16UpperLimit (Value determining the upper limit threshold)"
      mask help: Upper limit function in 16-bit fixed-point fractional implementation. Refer to the AMMCLIB User's Guide for further details.
      mask init:
      | if ~evalin('base','exist(''tS8'',''var'')')
      |   if (2 ~= exist('SWLIBS_Typedefs.mat','file'))
      |       error('File SWLIBS_Typedefs.mat is not on the Matlab path. Please add the AMMCLIB "bam" folder in the Matlab Search Path.');
      |   else
      |       evalin('base', 'load(''SWLIBS_Typedefs.mat'')');
      |   end
      | end
      | if showStates == 1
      |     % hidden state variables
      |     if strcmp(get_param([gcb '/f16UpperLimit'], 'BlockType'), 'Inport')
      |         posblk = get_param(gcb, 'Position');
      | 
      |         pos = get_param(    [gcb, '/f16UpperLimit'], 'Position');
      |         orient = get_param( [gcb, '/f16UpperLimit'], 'Orientation');
      |         delete_block(       [gcb, '/f16UpperLimit']);
      |         add_block('built-in/Ground', [gcb, '/f16UpperLimit'], 'Position', pos, 'Orientation', orient);
      | 
      | 
      | 
      |         set_param([gcb '/f16In'], 'Port', '1');
      | 
      |         set_param([gcb '/f16Out'], 'Port', '1');
      | 
      |         set_param(gcb,'MaskEnables',{'on','on'});
      | 
      |         if (posblk(4) - posblk(2)) > 50
      |           height = 50;
      |           set_param(gcb,'Position',[posblk(1), posblk(2), posblk(3), posblk(2)+height])
      |         end
      |     end
      | else
      |     % shown state variables
      |     if strcmp(get_param([gcb '/f16UpperLimit'], 'BlockType'), 'Ground')
      |         posblk = get_param(gcb, 'Position');
      | 
      |         pos = get_param(    [gcb, '/f16UpperLimit'], 'Position');
      |         orient = get_param( [gcb, '/f16UpperLimit'], 'Orientation');
      |         delete_block(       [gcb, '/f16UpperLimit']);
      |         add_block('built-in/Inport', [gcb, '/f16UpperLimit'], 'Position', pos, 'Orientation', orient, 'OutDataTypeStr', 'int16');
      | 
      | 
      | 
      |         set_param([gcb '/f16In'], 'Port', '1');
      |         set_param([gcb '/f16UpperLimit'], 'Port', '2');
      | 
      |         set_param([gcb '/f16Out'], 'Port', '1');
      | 
      |         set_param(gcb,'MaskEnables',{'on','off'});
      | 
      |         if (posblk(4) - posblk(2)) < 75
      |           height = 75;
      |           set_param(gcb,'Position',[posblk(1), posblk(2), posblk(3), posblk(2)+height])
      |         end
      |     end
      | end
      settings: RTWSystemCode=Inline
      mask TypeOptions showStates: Hide (faster execution) | Show (allows debugging; connect feedback loops manually)
      mask Callback showStates:
      | maskStr = get_param(gcb,'showStates');
      | if strcmp(maskStr,'Hide (faster execution)'),
      |     set_param(gcb,'MaskEnables',{'on','on'});
      | else
      |     set_param(gcb,'MaskEnables',{'on','off'});
      | end
      mask Display:
      | color('black');
      | pos = get_param(gcb, 'Position');
      | width = pos(3) - pos(1);
      | height = pos(4) - pos(2);
      | tX=width/2;
      | tY=height - 8;
      | color('black');
      | text(tX,tY, 'GFLIB_UpperLimit_F16', 'horizontalAlignment', 'center');
      | if showStates == 2
      |   color('red');
      |   text(tX,tY - 20, ['debugging mode' char(13) char(10) '(limited performance)'], 'horizontalAlignment', 'center');
      | end
  GFLIB_VMin_F16 : Subsystem  TreatAsAtomicUnit=on  mask(GFLIB_VMin_F16){}
      mask help: 16-bit fixed-point implementation of the GFLIB_VMin function, which finds the index of a vector minimum. Refer to the AMMCLIB User's Guide for further details.
      mask init: same as ammclib_bam/GDFLIB/F16/GDFLIB_FilterFIR_F16
      settings: RTWSystemCode=Inline
      mask Display: pos = get_param(gcb, 'Position');width = pos(3) - pos(1); height = pos(4) - pos(2);tX=width/2;tY=height - 8;color('black');text(tX,tY, 'GFLIB_VMin_F16', 'horizontalAlignment', 'center');
  GFLIB_VectorLimit_F16 : Subsystem  TreatAsAtomicUnit=on  mask(GFLIB_VectorLimit_F16){showStates=Hide (faster execution), f16Limit=0}
      mask prompts: showStates "Show internal states"; f16Limit "f16Limit (The maximum magnitude of the input 2-element vector)"
      mask help: 16-bit fixed-point fractional implementation of the GFLIB_VectorLimit function which limits the magnitude of the input 2-element vector, keeping its direction unchanged. Refer to the AMMCLIB User's Guide for further details.
      mask init:
      | if ~evalin('base','exist(''tS8'',''var'')')
      |   if (2 ~= exist('SWLIBS_Typedefs.mat','file'))
      |       error('File SWLIBS_Typedefs.mat is not on the Matlab path. Please add the AMMCLIB "bam" folder in the Matlab Search Path.');
      |   else
      |       evalin('base', 'load(''SWLIBS_Typedefs.mat'')');
      |   end
      | end
      | if showStates == 1
      |     % hidden state variables
      |     if strcmp(get_param([gcb '/f16Limit'], 'BlockType'), 'Inport')
      |         posblk = get_param(gcb, 'Position');
      | 
      |         pos = get_param(    [gcb, '/f16Limit'], 'Position');
      |         orient = get_param( [gcb, '/f16Limit'], 'Orientation');
      |         delete_block(       [gcb, '/f16Limit']);
      |         add_block('built-in/Ground', [gcb, '/f16Limit'], 'Position', pos, 'Orientation', orient);
      | 
      | 
      | 
      |         set_param([gcb '/pIn'], 'Port', '1');
      | 
      |         set_param([gcb '/bFlag'], 'Port', '1');
      |         set_param([gcb '/pOut'], 'Port', '2');
      | 
      |         set_param(gcb,'MaskEnables',{'on','on'});
      | 
      |         if (posblk(4) - posblk(2)) > 75
      |           height = 75;
      |           set_param(gcb,'Position',[posblk(1), posblk(2), posblk(3), posblk(2)+height])
      |         end
      |     end
      | else
      |     % shown state variables
      |     if strcmp(get_param([gcb '/f16Limit'], 'BlockType'), 'Ground')
      |         posblk = get_param(gcb, 'Position');
      | 
      |         pos = get_param(    [gcb, '/f16Limit'], 'Position');
      |         orient = get_param( [gcb, '/f16Limit'], 'Orientation');
      |         delete_block(       [gcb, '/f16Limit']);
      |         add_block('built-in/Inport', [gcb, '/f16Limit'], 'Position', pos, 'Orientation', orient, 'OutDataTypeStr', 'int16');
      | 
      | 
      | 
      |         set_param([gcb '/pIn'], 'Port', '1');
      |         set_param([gcb '/f16Limit'], 'Port', '2');
      | 
      |         set_param([gcb '/bFlag'], 'Port', '1');
      |         set_param([gcb '/pOut'], 'Port', '2');
      | 
      |         set_param(gcb,'MaskEnables',{'on','off'});
      | 
      |         if (posblk(4) - posblk(2)) < 75
      |           height = 75;
      |           set_param(gcb,'Position',[posblk(1), posblk(2), posblk(3), posblk(2)+height])
      |         end
      |     end
      | end
      settings: RTWSystemCode=Inline
      mask TypeOptions showStates: Hide (faster execution) | Show (allows debugging; connect feedback loops manually)
      mask Callback showStates:
      | maskStr = get_param(gcb,'showStates');
      | if strcmp(maskStr,'Hide (faster execution)'),
      |     set_param(gcb,'MaskEnables',{'on','on'});
      | else
      |     set_param(gcb,'MaskEnables',{'on','off'});
      | end
      mask Display:
      | color('black');
      | pos = get_param(gcb, 'Position');
      | width = pos(3) - pos(1);
      | height = pos(4) - pos(2);
      | tX=width/2;
      | tY=height - 8;
      | color('black');
      | text(tX,tY, 'GFLIB_VectorLimit_F16', 'horizontalAlignment', 'center');
      | if showStates == 2
      |   color('red');
      |   text(tX,tY - 20, ['debugging mode' char(13) char(10) '(limited performance)'], 'horizontalAlignment', 'center');
      | end
